simulink model "c00011M_harness"  (R2018a)
settings: Solver=FixedStepAuto  StartTime=0.0  StopTime=300  FixedStep=0.1  RelTol=1e-3
undefined symbols (not defined in the file): A1, hmax, PriorityTank, R1, R2, sigbuilder_block
(part 1 of 73)
settings Model: Creator=aarrieta  LastModifiedBy=umarkiegi

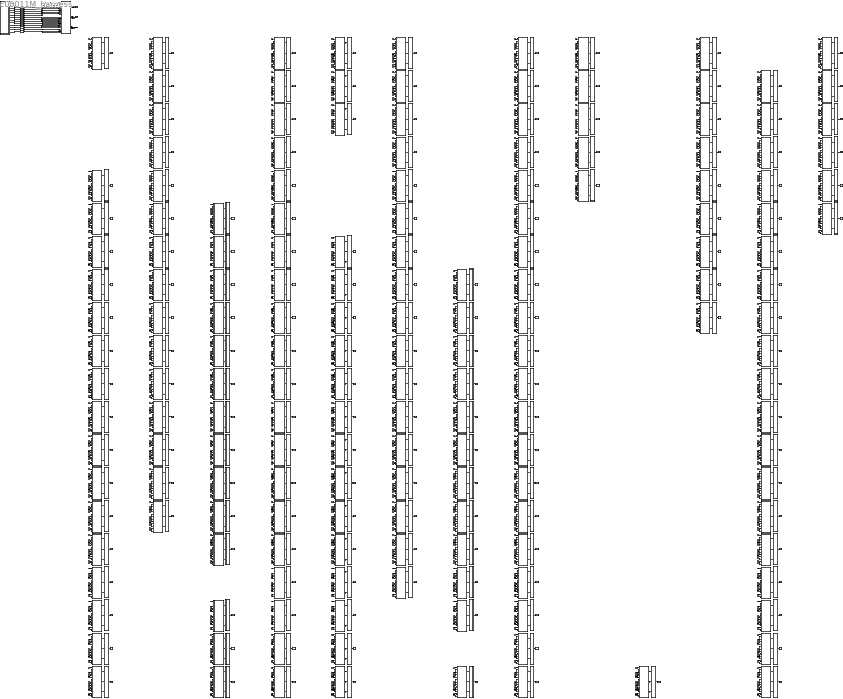
== system c00011M_harness ==
  CPSUT : Subsystem
  Eval : Subsystem
  Eval10 : Subsystem
  Eval100 : Subsystem
  Eval101 : Subsystem
  Eval102 : Subsystem
  Eval103 : Subsystem
  Eval104 : Subsystem
  Eval105 : Subsystem
  Eval106 : Subsystem
  Eval107 : Subsystem
  Eval108 : Subsystem
  Eval109 : Subsystem
  Eval11 : Subsystem
  Eval110 : Subsystem
  Eval111 : Subsystem
  Eval112 : Subsystem
  Eval113 : Subsystem
  Eval114 : Subsystem
  Eval115 : Subsystem
  Eval116 : Subsystem
  Eval12 : Subsystem
  Eval127 : Subsystem
  Eval128 : Subsystem
  Eval129 : Subsystem
  Eval13 : Subsystem
  Eval130 : Subsystem
  Eval131 : Subsystem
  Eval132 : Subsystem
  Eval133 : Subsystem
  Eval134 : Subsystem
  Eval135 : Subsystem
  Eval136 : Subsystem
  Eval137 : Subsystem
  Eval139 : Subsystem
  Eval14 : Subsystem
  Eval140 : Subsystem
  Eval141 : Subsystem
  Eval142 : Subsystem
  Eval143 : Subsystem
  Eval144 : Subsystem
  Eval145 : Subsystem
  Eval146 : Subsystem
  Eval147 : Subsystem
  Eval148 : Subsystem
  Eval149 : Subsystem
  Eval15 : Subsystem
  Eval150 : Subsystem
  Eval151 : Subsystem
  Eval152 : Subsystem
  Eval153 : Subsystem
  Eval154 : Subsystem
  Eval155 : Subsystem
  Eval156 : Subsystem
  Eval157 : Subsystem
  Eval158 : Subsystem
  Eval159 : Subsystem
  Eval16 : Subsystem
  Eval160 : Subsystem
  Eval161 : Subsystem
  Eval162 : Subsystem
  Eval163 : Subsystem
  Eval164 : Subsystem
  Eval17 : Subsystem
  Eval18 : Subsystem
  Eval19 : Subsystem
  Eval199 : Subsystem
  Eval20 : Subsystem
  Eval200 : Subsystem
  Eval201 : Subsystem
  Eval202 : Subsystem
  Eval203 : Subsystem
  Eval204 : Subsystem
  Eval205 : Subsystem
  Eval206 : Subsystem
  Eval207 : Subsystem
  Eval208 : Subsystem
  Eval21 : Subsystem
  Eval22 : Subsystem
  Eval221 : Subsystem
  Eval222 : Subsystem
  Eval223 : Subsystem
  Eval224 : Subsystem
  Eval225 : Subsystem
  Eval226 : Subsystem
  Eval227 : Subsystem
  Eval228 : Subsystem
  Eval229 : Subsystem
  Eval23 : Subsystem
  Eval230 : Subsystem
  Eval231 : Subsystem
  Eval232 : Subsystem
  Eval233 : Subsystem
  Eval234 : Subsystem
  Eval235 : Subsystem
  Eval236 : Subsystem
  Eval237 : Subsystem
  Eval238 : Subsystem
  Eval239 : Subsystem
  Eval24 : Subsystem
  Eval240 : Subsystem
  Eval241 : Subsystem
  Eval242 : Subsystem
  Eval243 : Subsystem
  Eval244 : Subsystem
  Eval245 : Subsystem
  Eval25 : Subsystem
  Eval26 : Subsystem
  Eval27 : Subsystem
  Eval28 : Subsystem
  Eval29 : Subsystem
  Eval30 : Subsystem
  Eval31 : Subsystem
  Eval32 : Subsystem
  Eval33 : Subsystem
  Eval34 : Subsystem
  Eval4 : Subsystem
  Eval45 : Subsystem
  Eval46 : Subsystem
  Eval47 : Subsystem
  Eval48 : Subsystem
  Eval49 : Subsystem
  Eval5 : Subsystem
  Eval50 : Subsystem
  Eval51 : Subsystem
  Eval52 : Subsystem
  Eval53 : Subsystem
  Eval54 : Subsystem
  Eval55 : Subsystem
  Eval57 : Subsystem
  Eval58 : Subsystem
  Eval59 : Subsystem
  Eval6 : Subsystem
  Eval60 : Subsystem
  Eval61 : Subsystem
  Eval62 : Subsystem
  Eval63 : Subsystem
  Eval64 : Subsystem
  Eval65 : Subsystem
  Eval66 : Subsystem
  Eval67 : Subsystem
  Eval68 : Subsystem
  Eval69 : Subsystem
  Eval7 : Subsystem
  Eval70 : Subsystem
  Eval71 : Subsystem
  Eval72 : Subsystem
  Eval73 : Subsystem
  Eval74 : Subsystem
  Eval75 : Subsystem
  Eval76 : Subsystem
  Eval77 : Subsystem
  Eval78 : Subsystem
  Eval79 : Subsystem
  Eval8 : Subsystem
  Eval80 : Subsystem
  Eval81 : Subsystem
  Eval82 : Subsystem
  Eval86 : Subsystem
  Eval87 : Subsystem
  Eval88 : Subsystem
  Eval89 : Subsystem
  Eval9 : Subsystem
  Eval90 : Subsystem
  Eval91 : Subsystem
  Eval92 : Subsystem
  Eval93 : Subsystem
  Eval94 : Subsystem
  Eval95 : Subsystem
  Eval96 : Subsystem
  Eval97 : Subsystem
  Eval98 : Subsystem
  Eval99 : Subsystem
  Inputs : Subsystem  Tag=STV Subsys  LoadFcn=sigbuilder_block('load');  StartFcn=sigbuilder_block('start');  StopFcn=sigbuilder_block('stop');  ClipboardFcn=sigbuilder_block('clipboard');  mask(Sigbuilder block){tuvar=[0:10]}
      mask init:
      | if ~strcmp(get_param(bdroot(gcb),'SimulationStatus'),'stopped'),tuvar = sigbuilder_block('maskInit'); end
      settings: CopyFcn=sigbuilder_block('copy');  DeleteFcn=sigbuilder_block('delete');  ModelCloseFcn=sigbuilder_block('modelClose');  PreSaveFcn=sigbuilder_block('preSave');  PauseFcn=sigbuilder_block('pause');  ContinueFcn=sigbuilder_block('continue');  NameChangeFcn=sigbuilder_block('namechange');  OpenFcn=sigbuilder_block('open',[276.75 163.5 675.75 486.75 ]);  CloseFcn=sigbuilder_block('close');
      mask Display: plot(0, 0, 100, 100,[2, 2, 32, 32, 2], [68, 8, 8, 68, 68],[32, 2], [38, 38], [32, 19, 2],[53, 60, 44], [32, 17, 17, 2],[16, 16, 31, 31]);txt = getActiveGroup(gcbh);text(2, 100, txt,'verticalAlignment', 'top');
  M001 : Subsystem
  M005 : Subsystem
  M006 : Subsystem
  M007 : Subsystem
  M008 : Subsystem
  M009 : Subsystem
  M010 : Subsystem
  M011 : Subsystem
  M012 : Subsystem
  M013 : Subsystem
  M014 : Subsystem
  M015 : Subsystem
  M016 : Subsystem
  M017 : Subsystem
  M018 : Subsystem
  M019 : Subsystem
  M020 : Subsystem
  M021 : Subsystem
  M022 : Subsystem
  M023 : Subsystem
  M024 : Subsystem
  M025 : Subsystem
  M026 : Subsystem
  M027 : Subsystem
  M028 : Subsystem
  M029 : Subsystem
  M030 : Subsystem
  M031 : Subsystem
  M032 : Subsystem
  M033 : Subsystem
  M034 : Subsystem
  M035 : Subsystem
  M046 : Subsystem
  M047 : Subsystem
  M048 : Subsystem
  M049 : Subsystem
  M050 : Subsystem
  M051 : Subsystem
  M052 : Subsystem
  M053 : Subsystem
  M054 : Subsystem
  M055 : Subsystem
  M056 : Subsystem
  M058 : Subsystem
  M059 : Subsystem
  M060 : Subsystem
  M061 : Subsystem
  M062 : Subsystem
  M063 : Subsystem
  M064 : Subsystem
  M065 : Subsystem
  M066 : Subsystem
  M067 : Subsystem
  M068 : Subsystem
  M069 : Subsystem
  M070 : Subsystem
  M071 : Subsystem
  M072 : Subsystem
  M073 : Subsystem
  M074 : Subsystem
  M075 : Subsystem
  M076 : Subsystem
  M077 : Subsystem
  M078 : Subsystem
  M079 : Subsystem
  M080 : Subsystem
  M081 : Subsystem
  M082 : Subsystem
  M083 : Subsystem
  M087 : Subsystem
  M088 : Subsystem
  M089 : Subsystem
  M090 : Subsystem
  M091 : Subsystem
  M092 : Subsystem
  M093 : Subsystem
  M094 : Subsystem
  M095 : Subsystem
  M096 : Subsystem
  M097 : Subsystem
  M098 : Subsystem
  M099 : Subsystem
  M100 : Subsystem
  M101 : Subsystem
  M102 : Subsystem
  M103 : Subsystem
  M104 : Subsystem
  M105 : Subsystem
  M106 : Subsystem
  M107 : Subsystem
  M108 : Subsystem
  M109 : Subsystem
  M110 : Subsystem
  M111 : Subsystem
  M112 : Subsystem
  M113 : Subsystem
  M114 : Subsystem
  M115 : Subsystem
  M116 : Subsystem
  M117 : Subsystem
  M128 : Subsystem
  M129 : Subsystem
  M130 : Subsystem
  M131 : Subsystem
  M132 : Subsystem
  M133 : Subsystem
  M134 : Subsystem
  M135 : Subsystem
  M136 : Subsystem
  M137 : Subsystem
  M138 : Subsystem
  M140 : Subsystem
  M141 : Subsystem
  M142 : Subsystem
  M143 : Subsystem
  M144 : Subsystem
  M145 : Subsystem
  M146 : Subsystem
  M147 : Subsystem
  M148 : Subsystem
  M149 : Subsystem
  M150 : Subsystem
  M151 : Subsystem
  M152 : Subsystem
  M153 : Subsystem
  M154 : Subsystem
  M155 : Subsystem
  M156 : Subsystem
  M157 : Subsystem
  M158 : Subsystem
  M159 : Subsystem
  M160 : Subsystem
  M161 : Subsystem
  M162 : Subsystem
  M163 : Subsystem
  M164 : Subsystem
  M165 : Subsystem
  M200 : Subsystem
  M201 : Subsystem
  M202 : Subsystem
  M203 : Subsystem
  M204 : Subsystem
  M205 : Subsystem
  M206 : Subsystem
  M207 : Subsystem
  M208 : Subsystem
  M209 : Subsystem
  M222 : Subsystem
  M223 : Subsystem
  M224 : Subsystem
  M225 : Subsystem
  M226 : Subsystem
  M227 : Subsystem
  M228 : Subsystem
  M229 : Subsystem
  M230 : Subsystem
  M231 : Subsystem
  M232 : Subsystem
  M233 : Subsystem
  M234 : Subsystem
  M235 : Subsystem
  M236 : Subsystem
  M237 : Subsystem
  M238 : Subsystem
  M239 : Subsystem
  M240 : Subsystem
  M241 : Subsystem
  M242 : Subsystem
  M243 : Subsystem
  M244 : Subsystem
  M245 : Subsystem
  M246 : Subsystem
  To Workspace : ToWorkspace  VariableName=mutant001  SampleTime=-1
  To Workspace10 : ToWorkspace  VariableName=mutant011  SampleTime=-1
  To Workspace100 : ToWorkspace  VariableName=mutant101  SampleTime=-1
  To Workspace101 : ToWorkspace  VariableName=mutant102  SampleTime=-1
  To Workspace102 : ToWorkspace  VariableName=mutant103  SampleTime=-1
  To Workspace103 : ToWorkspace  VariableName=mutant104  SampleTime=-1
  To Workspace104 : ToWorkspace  VariableName=mutant105  SampleTime=-1
  To Workspace105 : ToWorkspace  VariableName=mutant106  SampleTime=-1
  To Workspace106 : ToWorkspace  VariableName=mutant107  SampleTime=-1
  To Workspace107 : ToWorkspace  VariableName=mutant108  SampleTime=-1
  To Workspace108 : ToWorkspace  VariableName=mutant109  SampleTime=-1
  To Workspace109 : ToWorkspace  VariableName=mutant110  SampleTime=-1
  To Workspace11 : ToWorkspace  VariableName=mutant012  SampleTime=-1
  To Workspace110 : ToWorkspace  VariableName=mutant111  SampleTime=-1
  To Workspace111 : ToWorkspace  VariableName=mutant112  SampleTime=-1
  To Workspace112 : ToWorkspace  VariableName=mutant113  SampleTime=-1
  To Workspace113 : ToWorkspace  VariableName=mutant114  SampleTime=-1
  To Workspace114 : ToWorkspace  VariableName=mutant115  SampleTime=-1
  To Workspace115 : ToWorkspace  VariableName=mutant116  SampleTime=-1
  To Workspace116 : ToWorkspace  VariableName=mutant117  SampleTime=-1
  To Workspace12 : ToWorkspace  VariableName=mutant013  SampleTime=-1
  To Workspace127 : ToWorkspace  VariableName=mutant128  SampleTime=-1
  To Workspace128 : ToWorkspace  VariableName=mutant129  SampleTime=-1
  To Workspace129 : ToWorkspace  VariableName=mutant130  SampleTime=-1
  To Workspace13 : ToWorkspace  VariableName=mutant014  SampleTime=-1
  To Workspace130 : ToWorkspace  VariableName=mutant131  SampleTime=-1
  To Workspace131 : ToWorkspace  VariableName=mutant132  SampleTime=-1
  To Workspace132 : ToWorkspace  VariableName=mutant133  SampleTime=-1
  To Workspace133 : ToWorkspace  VariableName=mutant134  SampleTime=-1
  To Workspace134 : ToWorkspace  VariableName=mutant135  SampleTime=-1
  To Workspace135 : ToWorkspace  VariableName=mutant136  SampleTime=-1
  To Workspace136 : ToWorkspace  VariableName=mutant137  SampleTime=-1
  To Workspace137 : ToWorkspace  VariableName=mutant138  SampleTime=-1
  To Workspace139 : ToWorkspace  VariableName=mutant140  SampleTime=-1
  To Workspace14 : ToWorkspace  VariableName=mutant015  SampleTime=-1
  To Workspace140 : ToWorkspace  VariableName=mutant141  SampleTime=-1
  To Workspace141 : ToWorkspace  VariableName=mutant142  SampleTime=-1
  To Workspace142 : ToWorkspace  VariableName=mutant143  SampleTime=-1
  To Workspace143 : ToWorkspace  VariableName=mutant144  SampleTime=-1
  To Workspace144 : ToWorkspace  VariableName=mutant145  SampleTime=-1
  To Workspace145 : ToWorkspace  VariableName=mutant146  SampleTime=-1
  To Workspace146 : ToWorkspace  VariableName=mutant147  SampleTime=-1
  To Workspace147 : ToWorkspace  VariableName=mutant148  SampleTime=-1
  To Workspace148 : ToWorkspace  VariableName=mutant149  SampleTime=-1
  To Workspace149 : ToWorkspace  VariableName=mutant150  SampleTime=-1
  To Workspace15 : ToWorkspace  VariableName=mutant016  SampleTime=-1
  To Workspace150 : ToWorkspace  VariableName=mutant151  SampleTime=-1
  To Workspace151 : ToWorkspace  VariableName=mutant152  SampleTime=-1
  To Workspace152 : ToWorkspace  VariableName=mutant153  SampleTime=-1
  To Workspace153 : ToWorkspace  VariableName=mutant154  SampleTime=-1
  To Workspace154 : ToWorkspace  VariableName=mutant155  SampleTime=-1
  To Workspace155 : ToWorkspace  VariableName=mutant156  SampleTime=-1
  To Workspace156 : ToWorkspace  VariableName=mutant157  SampleTime=-1
  To Workspace157 : ToWorkspace  VariableName=mutant158  SampleTime=-1
  To Workspace158 : ToWorkspace  VariableName=mutant159  SampleTime=-1
  To Workspace159 : ToWorkspace  VariableName=mutant160  SampleTime=-1
  To Workspace16 : ToWorkspace  VariableName=mutant017  SampleTime=-1
  To Workspace160 : ToWorkspace  VariableName=mutant161  SampleTime=-1
  To Workspace161 : ToWorkspace  VariableName=mutant162  SampleTime=-1
  To Workspace162 : ToWorkspace  VariableName=mutant163  SampleTime=-1
  To Workspace163 : ToWorkspace  VariableName=mutant164  SampleTime=-1
  To Workspace164 : ToWorkspace  VariableName=mutant165  SampleTime=-1
  To Workspace17 : ToWorkspace  VariableName=mutant018  SampleTime=-1
  To Workspace18 : ToWorkspace  VariableName=mutant019  SampleTime=-1
  To Workspace19 : ToWorkspace  VariableName=mutant020  SampleTime=-1
  To Workspace199 : ToWorkspace  VariableName=mutant200  SampleTime=-1
  To Workspace20 : ToWorkspace  VariableName=mutant021  SampleTime=-1
  To Workspace200 : ToWorkspace  VariableName=mutant201  SampleTime=-1
  To Workspace201 : ToWorkspace  VariableName=mutant202  SampleTime=-1
  To Workspace202 : ToWorkspace  VariableName=mutant203  SampleTime=-1
  To Workspace203 : ToWorkspace  VariableName=mutant204  SampleTime=-1
  To Workspace204 : ToWorkspace  VariableName=mutant205  SampleTime=-1
  To Workspace205 : ToWorkspace  VariableName=mutant206  SampleTime=-1
  To Workspace206 : ToWorkspace  VariableName=mutant207  SampleTime=-1
  To Workspace207 : ToWorkspace  VariableName=mutant208  SampleTime=-1
  To Workspace208 : ToWorkspace  VariableName=mutant209  SampleTime=-1
  To Workspace21 : ToWorkspace  VariableName=mutant022  SampleTime=-1
  To Workspace22 : ToWorkspace  VariableName=mutant023  SampleTime=-1
  To Workspace221 : ToWorkspace  VariableName=mutant222  SampleTime=-1
  To Workspace222 : ToWorkspace  VariableName=mutant223  SampleTime=-1
  To Workspace223 : ToWorkspace  VariableName=mutant224  SampleTime=-1
  To Workspace224 : ToWorkspace  VariableName=mutant225  SampleTime=-1
  To Workspace225 : ToWorkspace  VariableName=mutant226  SampleTime=-1
  To Workspace226 : ToWorkspace  VariableName=mutant227  SampleTime=-1
  To Workspace227 : ToWorkspace  VariableName=mutant228  SampleTime=-1
  To Workspace228 : ToWorkspace  VariableName=mutant229  SampleTime=-1
  To Workspace229 : ToWorkspace  VariableName=mutant230  SampleTime=-1
  To Workspace23 : ToWorkspace  VariableName=mutant024  SampleTime=-1
  To Workspace230 : ToWorkspace  VariableName=mutant231  SampleTime=-1
  To Workspace231 : ToWorkspace  VariableName=mutant232  SampleTime=-1
  To Workspace232 : ToWorkspace  VariableName=mutant233  SampleTime=-1
  To Workspace233 : ToWorkspace  VariableName=mutant234  SampleTime=-1
  To Workspace234 : ToWorkspace  VariableName=mutant235  SampleTime=-1
  To Workspace235 : ToWorkspace  VariableName=mutant236  SampleTime=-1
  To Workspace236 : ToWorkspace  VariableName=mutant237  SampleTime=-1
  To Workspace237 : ToWorkspace  VariableName=mutant238  SampleTime=-1
  To Workspace238 : ToWorkspace  VariableName=mutant239  SampleTime=-1
  To Workspace239 : ToWorkspace  VariableName=mutant240  SampleTime=-1
  To Workspace24 : ToWorkspace  VariableName=mutant025  SampleTime=-1
  To Workspace240 : ToWorkspace  VariableName=mutant241  SampleTime=-1
  To Workspace241 : ToWorkspace  VariableName=mutant242  SampleTime=-1
  To Workspace242 : ToWorkspace  VariableName=mutant243  SampleTime=-1
  To Workspace243 : ToWorkspace  VariableName=mutant244  SampleTime=-1
  To Workspace244 : ToWorkspace  VariableName=mutant245  SampleTime=-1
  To Workspace245 : ToWorkspace  VariableName=mutant246  SampleTime=-1
  To Workspace25 : ToWorkspace  VariableName=mutant026  SampleTime=-1
  To Workspace26 : ToWorkspace  VariableName=mutant027  SampleTime=-1
  To Workspace27 : ToWorkspace  VariableName=mutant028  SampleTime=-1
  To Workspace28 : ToWorkspace  VariableName=mutant029  SampleTime=-1
  To Workspace29 : ToWorkspace  VariableName=mutant030  SampleTime=-1
  To Workspace30 : ToWorkspace  VariableName=mutant031  SampleTime=-1
  To Workspace31 : ToWorkspace  VariableName=mutant032  SampleTime=-1
  To Workspace32 : ToWorkspace  VariableName=mutant033  SampleTime=-1
  To Workspace33 : ToWorkspace  VariableName=mutant034  SampleTime=-1
  To Workspace34 : ToWorkspace  VariableName=mutant035  SampleTime=-1
  To Workspace4 : ToWorkspace  VariableName=mutant005  SampleTime=-1
  To Workspace45 : ToWorkspace  VariableName=mutant046  SampleTime=-1
  To Workspace46 : ToWorkspace  VariableName=mutant047  SampleTime=-1
  To Workspace47 : ToWorkspace  VariableName=mutant048  SampleTime=-1
  To Workspace48 : ToWorkspace  VariableName=mutant049  SampleTime=-1
  To Workspace49 : ToWorkspace  VariableName=mutant050  SampleTime=-1
  To Workspace5 : ToWorkspace  VariableName=mutant006  SampleTime=-1
  To Workspace50 : ToWorkspace  VariableName=mutant051  SampleTime=-1
  To Workspace51 : ToWorkspace  VariableName=mutant052  SampleTime=-1
  To Workspace52 : ToWorkspace  VariableName=mutant053  SampleTime=-1
  To Workspace53 : ToWorkspace  VariableName=mutant054  SampleTime=-1
  To Workspace54 : ToWorkspace  VariableName=mutant055  SampleTime=-1
  To Workspace55 : ToWorkspace  VariableName=mutant056  SampleTime=-1
  To Workspace57 : ToWorkspace  VariableName=mutant058  SampleTime=-1
  To Workspace58 : ToWorkspace  VariableName=mutant059  SampleTime=-1
  To Workspace59 : ToWorkspace  VariableName=mutant060  SampleTime=-1
  To Workspace6 : ToWorkspace  VariableName=mutant007  SampleTime=-1
  To Workspace60 : ToWorkspace  VariableName=mutant061  SampleTime=-1
  To Workspace61 : ToWorkspace  VariableName=mutant062  SampleTime=-1
  To Workspace62 : ToWorkspace  VariableName=mutant063  SampleTime=-1
  To Workspace63 : ToWorkspace  VariableName=mutant064  SampleTime=-1
  To Workspace64 : ToWorkspace  VariableName=mutant065  SampleTime=-1
  To Workspace65 : ToWorkspace  VariableName=mutant066  SampleTime=-1
  To Workspace66 : ToWorkspace  VariableName=mutant067  SampleTime=-1
  To Workspace67 : ToWorkspace  VariableName=mutant068  SampleTime=-1
  To Workspace68 : ToWorkspace  VariableName=mutant069  SampleTime=-1
  To Workspace69 : ToWorkspace  VariableName=mutant070  SampleTime=-1
  To Workspace7 : ToWorkspace  VariableName=mutant008  SampleTime=-1
  To Workspace70 : ToWorkspace  VariableName=mutant071  SampleTime=-1
  To Workspace71 : ToWorkspace  VariableName=mutant072  SampleTime=-1
  To Workspace72 : ToWorkspace  VariableName=mutant073  SampleTime=-1
  To Workspace73 : ToWorkspace  VariableName=mutant074  SampleTime=-1
  To Workspace74 : ToWorkspace  VariableName=mutant075  SampleTime=-1
  To Workspace75 : ToWorkspace  VariableName=mutant076  SampleTime=-1
  To Workspace76 : ToWorkspace  VariableName=mutant077  SampleTime=-1
  To Workspace77 : ToWorkspace  VariableName=mutant078  SampleTime=-1
  To Workspace78 : ToWorkspace  VariableName=mutant079  SampleTime=-1
  To Workspace79 : ToWorkspace  VariableName=mutant080  SampleTime=-1
  To Workspace8 : ToWorkspace  VariableName=mutant009  SampleTime=-1
  To Workspace80 : ToWorkspace  VariableName=mutant081  SampleTime=-1
  To Workspace81 : ToWorkspace  VariableName=mutant082  SampleTime=-1
  To Workspace82 : ToWorkspace  VariableName=mutant083  SampleTime=-1
  To Workspace86 : ToWorkspace  VariableName=mutant087  SampleTime=-1
  To Workspace87 : ToWorkspace  VariableName=mutant088  SampleTime=-1
  To Workspace88 : ToWorkspace  VariableName=mutant089  SampleTime=-1
  To Workspace89 : ToWorkspace  VariableName=mutant090  SampleTime=-1
  To Workspace9 : ToWorkspace  VariableName=mutant010  SampleTime=-1
  To Workspace90 : ToWorkspace  VariableName=mutant091  SampleTime=-1
  To Workspace91 : ToWorkspace  VariableName=mutant092  SampleTime=-1
  To Workspace92 : ToWorkspace  VariableName=mutant093  SampleTime=-1
  To Workspace93 : ToWorkspace  VariableName=mutant094  SampleTime=-1
  To Workspace94 : ToWorkspace  VariableName=mutant095  SampleTime=-1
  To Workspace95 : ToWorkspace  VariableName=mutant096  SampleTime=-1
  To Workspace96 : ToWorkspace  VariableName=mutant097  SampleTime=-1
  To Workspace97 : ToWorkspace  VariableName=mutant098  SampleTime=-1
  To Workspace98 : ToWorkspace  VariableName=mutant099  SampleTime=-1
  To Workspace99 : ToWorkspace  VariableName=mutant100  SampleTime=-1
  dtc_CT1 : DataTypeConversion
  dtc_CT2 : DataTypeConversion
  dtc_CT3 : DataTypeConversion
  dtc_E3 : DataTypeConversion
  dtc_EB1 : DataTypeConversion
  dtc_EB2 : DataTypeConversion
  dtc_EB3 : DataTypeConversion
  dtc_F3 : DataTypeConversion
  dtc_MR1 : DataTypeConversion
  dtc_MR2 : DataTypeConversion
  dtc_T1 : DataTypeConversion
  dtc_T2 : DataTypeConversion
  dtc_T3 : DataTypeConversion
  LL1 : Outport
  LL2 : Outport  Port=2
  LL3 : Outport  Port=3
  tag scope: out1=global, out2=global, out3=global
  wires:
  CPSUT/1(LL1) -> [out1], LL1/1
  CPSUT/2(LL2) -> [out2], LL2/1
  CPSUT/3(LL3) -> [out3], LL3/1
  [in1] -> M001/1(CT1)
  [in4] -> M001/2(MR1)
  [in5] -> M001/3(T1)
  [in6] -> M001/4(EB1)
  [in7] -> M001/5(CT2)
  [in10] -> M001/6(MR2)
  [in11] -> M001/7(T2)
  [in12] -> M001/8(EB2)
  [in13] -> M001/9(CT3)
  [in14] -> M001/10(F3)
  [in15] -> M001/11(E3)
  [in17] -> M001/12(T3)
  [in18] -> M001/13(EB3)
  Eval/1(Out1) -> To Workspace/1
  M001/1(LL1) -> Eval/1(In1)
  M001/2(LL2) -> Eval/2(In2)
  M001/3(LL3) -> Eval/3(In3)
  [in1] -> M005/1(CT1)
  [in4] -> M005/2(MR1)
  [in5] -> M005/3(T1)
  [in6] -> M005/4(EB1)
  [in7] -> M005/5(CT2)
  [in10] -> M005/6(MR2)
  [in11] -> M005/7(T2)
  [in12] -> M005/8(EB2)
  [in13] -> M005/9(CT3)
  [in14] -> M005/10(F3)
  [in15] -> M005/11(E3)
  [in17] -> M005/12(T3)
  [in18] -> M005/13(EB3)
  M005/1(LL1) -> Eval4/1(In1)
  M005/2(LL2) -> Eval4/2(In2)
  M005/3(LL3) -> Eval4/3(In3)
  Eval4/1(Out1) -> To Workspace4/1
  [in1] -> M006/1(CT1)
  [in4] -> M006/2(MR1)
  [in5] -> M006/3(T1)
  [in6] -> M006/4(EB1)
  [in7] -> M006/5(CT2)
  [in10] -> M006/6(MR2)
  [in11] -> M006/7(T2)
  [in12] -> M006/8(EB2)
  [in13] -> M006/9(CT3)
  [in14] -> M006/10(F3)
  [in15] -> M006/11(E3)
  [in17] -> M006/12(T3)
  [in18] -> M006/13(EB3)
  M006/1(LL1) -> Eval5/1(In1)
  M006/2(LL2) -> Eval5/2(In2)
  M006/3(LL3) -> Eval5/3(In3)
  Eval5/1(Out1) -> To Workspace5/1
  [in1] -> M007/1(CT1)
  [in4] -> M007/2(MR1)
  [in5] -> M007/3(T1)
  [in6] -> M007/4(EB1)
  [in7] -> M007/5(CT2)
  [in10] -> M007/6(MR2)
  [in11] -> M007/7(T2)
  [in12] -> M007/8(EB2)
  [in13] -> M007/9(CT3)
  [in14] -> M007/10(F3)
  [in15] -> M007/11(E3)
  [in17] -> M007/12(T3)
  [in18] -> M007/13(EB3)
  M007/1(LL1) -> Eval6/1(In1)
  M007/2(LL2) -> Eval6/2(In2)
  M007/3(LL3) -> Eval6/3(In3)
  Eval6/1(Out1) -> To Workspace6/1
  [in1] -> M008/1(CT1)
  [in4] -> M008/2(MR1)
  [in5] -> M008/3(T1)
  [in6] -> M008/4(EB1)
  [in7] -> M008/5(CT2)
  [in10] -> M008/6(MR2)
  [in11] -> M008/7(T2)
  [in12] -> M008/8(EB2)
  [in13] -> M008/9(CT3)
  [in14] -> M008/10(F3)
  [in15] -> M008/11(E3)
  [in17] -> M008/12(T3)
  [in18] -> M008/13(EB3)
  M008/1(LL1) -> Eval7/1(In1)
  M008/2(LL2) -> Eval7/2(In2)
  M008/3(LL3) -> Eval7/3(In3)
  Eval7/1(Out1) -> To Workspace7/1
  [in1] -> M009/1(CT1)
  [in4] -> M009/2(MR1)
  [in5] -> M009/3(T1)
  [in6] -> M009/4(EB1)
  [in7] -> M009/5(CT2)
  [in10] -> M009/6(MR2)
  [in11] -> M009/7(T2)
  [in12] -> M009/8(EB2)
  [in13] -> M009/9(CT3)
  [in14] -> M009/10(F3)
  [in15] -> M009/11(E3)
  [in17] -> M009/12(T3)
  [in18] -> M009/13(EB3)
  M009/1(LL1) -> Eval8/1(In1)
  M009/2(LL2) -> Eval8/2(In2)
  M009/3(LL3) -> Eval8/3(In3)
  Eval8/1(Out1) -> To Workspace8/1
  [in1] -> M010/1(CT1)
  [in4] -> M010/2(MR1)
  [in5] -> M010/3(T1)
  [in6] -> M010/4(EB1)
  [in7] -> M010/5(CT2)
  [in10] -> M010/6(MR2)
  [in11] -> M010/7(T2)
  [in12] -> M010/8(EB2)
  [in13] -> M010/9(CT3)
  [in14] -> M010/10(F3)
  [in15] -> M010/11(E3)
  [in17] -> M010/12(T3)
  [in18] -> M010/13(EB3)
  M010/1(LL1) -> Eval9/1(In1)
  M010/2(LL2) -> Eval9/2(In2)
  M010/3(LL3) -> Eval9/3(In3)
  Eval9/1(Out1) -> To Workspace9/1
  [in1] -> M011/1(CT1)
  [in4] -> M011/2(MR1)
  [in5] -> M011/3(T1)
  [in6] -> M011/4(EB1)
  [in7] -> M011/5(CT2)
  [in10] -> M011/6(MR2)
  [in11] -> M011/7(T2)
  [in12] -> M011/8(EB2)
  [in13] -> M011/9(CT3)
  [in14] -> M011/10(F3)
  [in15] -> M011/11(E3)
  [in17] -> M011/12(T3)
  [in18] -> M011/13(EB3)
  M011/1(LL1) -> Eval10/1(In1)
  M011/2(LL2) -> Eval10/2(In2)
  M011/3(LL3) -> Eval10/3(In3)
  Eval10/1(Out1) -> To Workspace10/1
  [in1] -> M012/1(CT1)
  [in4] -> M012/2(MR1)
  [in5] -> M012/3(T1)
  [in6] -> M012/4(EB1)
  [in7] -> M012/5(CT2)
  [in10] -> M012/6(MR2)
  [in11] -> M012/7(T2)
  [in12] -> M012/8(EB2)
  [in13] -> M012/9(CT3)
  [in14] -> M012/10(F3)
  [in15] -> M012/11(E3)
  [in17] -> M012/12(T3)
  [in18] -> M012/13(EB3)
  M012/1(LL1) -> Eval11/1(In1)
  M012/2(LL2) -> Eval11/2(In2)
  M012/3(LL3) -> Eval11/3(In3)
  Eval11/1(Out1) -> To Workspace11/1
  [in1] -> M013/1(CT1)
  [in4] -> M013/2(MR1)
  [in5] -> M013/3(T1)
  [in6] -> M013/4(EB1)
  [in7] -> M013/5(CT2)
  [in10] -> M013/6(MR2)
  [in11] -> M013/7(T2)
  [in12] -> M013/8(EB2)
  [in13] -> M013/9(CT3)
  [in14] -> M013/10(F3)
  [in15] -> M013/11(E3)
  [in17] -> M013/12(T3)
  [in18] -> M013/13(EB3)
  M013/1(LL1) -> Eval12/1(In1)
  M013/2(LL2) -> Eval12/2(In2)
  M013/3(LL3) -> Eval12/3(In3)
  Eval12/1(Out1) -> To Workspace12/1
  [in1] -> M014/1(CT1)
  [in4] -> M014/2(MR1)
  [in5] -> M014/3(T1)
  [in6] -> M014/4(EB1)
  [in7] -> M014/5(CT2)
  [in10] -> M014/6(MR2)
  [in11] -> M014/7(T2)
  [in12] -> M014/8(EB2)
  [in13] -> M014/9(CT3)
  [in14] -> M014/10(F3)
  [in15] -> M014/11(E3)
  [in17] -> M014/12(T3)
  [in18] -> M014/13(EB3)
  M014/1(LL1) -> Eval13/1(In1)
  M014/2(LL2) -> Eval13/2(In2)
  M014/3(LL3) -> Eval13/3(In3)
  Eval13/1(Out1) -> To Workspace13/1
  [in1] -> M015/1(CT1)
  [in4] -> M015/2(MR1)
  [in5] -> M015/3(T1)
  [in6] -> M015/4(EB1)
  [in7] -> M015/5(CT2)
  [in10] -> M015/6(MR2)
  [in11] -> M015/7(T2)
  [in12] -> M015/8(EB2)
  [in13] -> M015/9(CT3)
  [in14] -> M015/10(F3)
  [in15] -> M015/11(E3)
  [in17] -> M015/12(T3)
  [in18] -> M015/13(EB3)
  M015/1(LL1) -> Eval14/1(In1)
  M015/2(LL2) -> Eval14/2(In2)
  M015/3(LL3) -> Eval14/3(In3)
  Eval14/1(Out1) -> To Workspace14/1
  [in1] -> M016/1(CT1)
  [in4] -> M016/2(MR1)
  [in5] -> M016/3(T1)
  [in6] -> M016/4(EB1)
  [in7] -> M016/5(CT2)
  [in10] -> M016/6(MR2)
  [in11] -> M016/7(T2)
  [in12] -> M016/8(EB2)
  [in13] -> M016/9(CT3)
  [in14] -> M016/10(F3)
  [in15] -> M016/11(E3)
  [in17] -> M016/12(T3)
  [in18] -> M016/13(EB3)
  M016/1(LL1) -> Eval15/1(In1)
  M016/2(LL2) -> Eval15/2(In2)
  M016/3(LL3) -> Eval15/3(In3)
  Eval15/1(Out1) -> To Workspace15/1
  [in1] -> M017/1(CT1)
  [in4] -> M017/2(MR1)
  [in5] -> M017/3(T1)
  [in6] -> M017/4(EB1)
  [in7] -> M017/5(CT2)
  [in10] -> M017/6(MR2)
  [in11] -> M017/7(T2)
  [in12] -> M017/8(EB2)
  [in13] -> M017/9(CT3)
  [in14] -> M017/10(F3)
  [in15] -> M017/11(E3)
  [in17] -> M017/12(T3)
  [in18] -> M017/13(EB3)
  M017/1(LL1) -> Eval16/1(In1)
  M017/2(LL2) -> Eval16/2(In2)
  M017/3(LL3) -> Eval16/3(In3)
  Eval16/1(Out1) -> To Workspace16/1
  [in1] -> M018/1(CT1)
  [in4] -> M018/2(MR1)
  [in5] -> M018/3(T1)
  [in6] -> M018/4(EB1)
  [in7] -> M018/5(CT2)
  [in10] -> M018/6(MR2)
  [in11] -> M018/7(T2)
  [in12] -> M018/8(EB2)
  [in13] -> M018/9(CT3)
  [in14] -> M018/10(F3)
  [in15] -> M018/11(E3)
  [in17] -> M018/12(T3)
  [in18] -> M018/13(EB3)
  M018/1(LL1) -> Eval17/1(In1)
  M018/2(LL2) -> Eval17/2(In2)
  M018/3(LL3) -> Eval17/3(In3)
  Eval17/1(Out1) -> To Workspace17/1
  [in1] -> M019/1(CT1)
  [in4] -> M019/2(MR1)
  [in5] -> M019/3(T1)
  [in6] -> M019/4(EB1)
  [in7] -> M019/5(CT2)
  [in10] -> M019/6(MR2)
  [in11] -> M019/7(T2)
  [in12] -> M019/8(EB2)
  [in13] -> M019/9(CT3)
  [in14] -> M019/10(F3)
  [in15] -> M019/11(E3)
  [in17] -> M019/12(T3)
  [in18] -> M019/13(EB3)
  M019/1(LL1) -> Eval18/1(In1)
  M019/2(LL2) -> Eval18/2(In2)
  M019/3(LL3) -> Eval18/3(In3)
  Eval18/1(Out1) -> To Workspace18/1
  [in1] -> M020/1(CT1)
  [in4] -> M020/2(MR1)
  [in5] -> M020/3(T1)
  [in6] -> M020/4(EB1)
  [in7] -> M020/5(CT2)
  [in10] -> M020/6(MR2)
  [in11] -> M020/7(T2)
  [in12] -> M020/8(EB2)
  [in13] -> M020/9(CT3)
  [in14] -> M020/10(F3)
  [in15] -> M020/11(E3)
  [in17] -> M020/12(T3)
  [in18] -> M020/13(EB3)
  M020/1(LL1) -> Eval19/1(In1)
  M020/2(LL2) -> Eval19/2(In2)
  M020/3(LL3) -> Eval19/3(In3)
  Eval19/1(Out1) -> To Workspace19/1
  [in1] -> M021/1(CT1)
  [in4] -> M021/2(MR1)
  [in5] -> M021/3(T1)
  [in6] -> M021/4(EB1)
  [in7] -> M021/5(CT2)
  [in10] -> M021/6(MR2)
  [in11] -> M021/7(T2)
  [in12] -> M021/8(EB2)
  [in13] -> M021/9(CT3)
  [in14] -> M021/10(F3)
  [in15] -> M021/11(E3)
  [in17] -> M021/12(T3)
  [in18] -> M021/13(EB3)
  M021/1(LL1) -> Eval20/1(In1)
  M021/2(LL2) -> Eval20/2(In2)
  M021/3(LL3) -> Eval20/3(In3)
  Eval20/1(Out1) -> To Workspace20/1
  [in1] -> M022/1(CT1)
  [in4] -> M022/2(MR1)
  [in5] -> M022/3(T1)
  [in6] -> M022/4(EB1)
  [in7] -> M022/5(CT2)
  [in10] -> M022/6(MR2)
  [in11] -> M022/7(T2)
  [in12] -> M022/8(EB2)
  [in13] -> M022/9(CT3)
  [in14] -> M022/10(F3)
  [in15] -> M022/11(E3)
  [in17] -> M022/12(T3)
  [in18] -> M022/13(EB3)
  M022/1(LL1) -> Eval21/1(In1)
  M022/2(LL2) -> Eval21/2(In2)
  M022/3(LL3) -> Eval21/3(In3)
  Eval21/1(Out1) -> To Workspace21/1
  [in1] -> M023/1(CT1)
  [in4] -> M023/2(MR1)
  [in5] -> M023/3(T1)
  [in6] -> M023/4(EB1)
  [in7] -> M023/5(CT2)
  [in10] -> M023/6(MR2)
  [in11] -> M023/7(T2)
  [in12] -> M023/8(EB2)
  [in13] -> M023/9(CT3)
  [in14] -> M023/10(F3)
  [in15] -> M023/11(E3)
  [in17] -> M023/12(T3)
  [in18] -> M023/13(EB3)
  M023/1(LL1) -> Eval22/1(In1)
  M023/2(LL2) -> Eval22/2(In2)
  M023/3(LL3) -> Eval22/3(In3)
  Eval22/1(Out1) -> To Workspace22/1
  [in1] -> M024/1(CT1)
  [in4] -> M024/2(MR1)
  [in5] -> M024/3(T1)
  [in6] -> M024/4(EB1)
  [in7] -> M024/5(CT2)
  [in10] -> M024/6(MR2)
  [in11] -> M024/7(T2)
  [in12] -> M024/8(EB2)
  [in13] -> M024/9(CT3)
  [in14] -> M024/10(F3)
  [in15] -> M024/11(E3)
  [in17] -> M024/12(T3)
  [in18] -> M024/13(EB3)
  M024/1(LL1) -> Eval23/1(In1)
  M024/2(LL2) -> Eval23/2(In2)
  M024/3(LL3) -> Eval23/3(In3)
  Eval23/1(Out1) -> To Workspace23/1
  [in1] -> M025/1(CT1)
  [in4] -> M025/2(MR1)
  [in5] -> M025/3(T1)
  [in6] -> M025/4(EB1)
  [in7] -> M025/5(CT2)
  [in10] -> M025/6(MR2)
  [in11] -> M025/7(T2)
  [in12] -> M025/8(EB2)
  [in13] -> M025/9(CT3)
  [in14] -> M025/10(F3)
  [in15] -> M025/11(E3)
  [in17] -> M025/12(T3)
  [in18] -> M025/13(EB3)
  M025/1(LL1) -> Eval24/1(In1)
  M025/2(LL2) -> Eval24/2(In2)
  M025/3(LL3) -> Eval24/3(In3)
  Eval24/1(Out1) -> To Workspace24/1
  [in1] -> M026/1(CT1)
  [in4] -> M026/2(MR1)
  [in5] -> M026/3(T1)
  [in6] -> M026/4(EB1)
  [in7] -> M026/5(CT2)
  [in10] -> M026/6(MR2)
  [in11] -> M026/7(T2)
  [in12] -> M026/8(EB2)
  [in13] -> M026/9(CT3)
  [in14] -> M026/10(F3)
  [in15] -> M026/11(E3)
  [in17] -> M026/12(T3)
  [in18] -> M026/13(EB3)
  M026/1(LL1) -> Eval25/1(In1)
  M026/2(LL2) -> Eval25/2(In2)
  M026/3(LL3) -> Eval25/3(In3)
  Eval25/1(Out1) -> To Workspace25/1
  [in1] -> M027/1(CT1)
  [in4] -> M027/2(MR1)
  [in5] -> M027/3(T1)
  [in6] -> M027/4(EB1)
  [in7] -> M027/5(CT2)
  [in10] -> M027/6(MR2)
  [in11] -> M027/7(T2)
  [in12] -> M027/8(EB2)
  [in13] -> M027/9(CT3)
  [in14] -> M027/10(F3)
  [in15] -> M027/11(E3)
  [in17] -> M027/12(T3)
  [in18] -> M027/13(EB3)
  M027/1(LL1) -> Eval26/1(In1)
  M027/2(LL2) -> Eval26/2(In2)
  M027/3(LL3) -> Eval26/3(In3)
  Eval26/1(Out1) -> To Workspace26/1
  [in1] -> M028/1(CT1)
  [in4] -> M028/2(MR1)
  [in5] -> M028/3(T1)
  [in6] -> M028/4(EB1)
  [in7] -> M028/5(CT2)
  [in10] -> M028/6(MR2)
  [in11] -> M028/7(T2)
  [in12] -> M028/8(EB2)
  [in13] -> M028/9(CT3)
  [in14] -> M028/10(F3)
  [in15] -> M028/11(E3)
  [in17] -> M028/12(T3)
  [in18] -> M028/13(EB3)
  M028/1(LL1) -> Eval27/1(In1)
  M028/2(LL2) -> Eval27/2(In2)
  M028/3(LL3) -> Eval27/3(In3)
  Eval27/1(Out1) -> To Workspace27/1
  [in1] -> M029/1(CT1)
  [in4] -> M029/2(MR1)
  [in5] -> M029/3(T1)
  [in6] -> M029/4(EB1)
  [in7] -> M029/5(CT2)
  [in10] -> M029/6(MR2)
  [in11] -> M029/7(T2)
  [in12] -> M029/8(EB2)
  [in13] -> M029/9(CT3)
  [in14] -> M029/10(F3)
  [in15] -> M029/11(E3)
  [in17] -> M029/12(T3)
  [in18] -> M029/13(EB3)
  M029/1(LL1) -> Eval28/1(In1)
  M029/2(LL2) -> Eval28/2(In2)
  M029/3(LL3) -> Eval28/3(In3)
  Eval28/1(Out1) -> To Workspace28/1
  [in1] -> M030/1(CT1)
  [in4] -> M030/2(MR1)
  [in5] -> M030/3(T1)
  [in6] -> M030/4(EB1)
  [in7] -> M030/5(CT2)
  [in10] -> M030/6(MR2)
  [in11] -> M030/7(T2)
  [in12] -> M030/8(EB2)
  [in13] -> M030/9(CT3)
  [in14] -> M030/10(F3)
  [in15] -> M030/11(E3)
  [in17] -> M030/12(T3)
  [in18] -> M030/13(EB3)
  M030/1(LL1) -> Eval29/1(In1)
  M030/2(LL2) -> Eval29/2(In2)
  M030/3(LL3) -> Eval29/3(In3)
  Eval29/1(Out1) -> To Workspace29/1
  [in1] -> M031/1(CT1)
  [in4] -> M031/2(MR1)
  [in5] -> M031/3(T1)
  [in6] -> M031/4(EB1)
  [in7] -> M031/5(CT2)
  [in10] -> M031/6(MR2)
  [in11] -> M031/7(T2)
  [in12] -> M031/8(EB2)
  [in13] -> M031/9(CT3)
  [in14] -> M031/10(F3)
  [in15] -> M031/11(E3)
  [in17] -> M031/12(T3)
  [in18] -> M031/13(EB3)
  M031/1(LL1) -> Eval30/1(In1)
  M031/2(LL2) -> Eval30/2(In2)
  M031/3(LL3) -> Eval30/3(In3)
  Eval30/1(Out1) -> To Workspace30/1
  [in1] -> M032/1(CT1)
  [in4] -> M032/2(MR1)
  [in5] -> M032/3(T1)
  [in6] -> M032/4(EB1)
  [in7] -> M032/5(CT2)
  [in10] -> M032/6(MR2)
  [in11] -> M032/7(T2)
  [in12] -> M032/8(EB2)
  [in13] -> M032/9(CT3)
  [in14] -> M032/10(F3)
  [in15] -> M032/11(E3)
  [in17] -> M032/12(T3)
  [in18] -> M032/13(EB3)
  M032/1(LL1) -> Eval31/1(In1)
  M032/2(LL2) -> Eval31/2(In2)
  M032/3(LL3) -> Eval31/3(In3)
  Eval31/1(Out1) -> To Workspace31/1
  [in1] -> M033/1(CT1)
  [in4] -> M033/2(MR1)
  [in5] -> M033/3(T1)
  [in6] -> M033/4(EB1)
  [in7] -> M033/5(CT2)
  [in10] -> M033/6(MR2)
  [in11] -> M033/7(T2)
  [in12] -> M033/8(EB2)
  [in13] -> M033/9(CT3)
  [in14] -> M033/10(F3)
  [in15] -> M033/11(E3)
  [in17] -> M033/12(T3)
  [in18] -> M033/13(EB3)
  M033/1(LL1) -> Eval32/1(In1)
  M033/2(LL2) -> Eval32/2(In2)
  M033/3(LL3) -> Eval32/3(In3)
  Eval32/1(Out1) -> To Workspace32/1
  [in1] -> M034/1(CT1)
  [in4] -> M034/2(MR1)
  [in5] -> M034/3(T1)
  [in6] -> M034/4(EB1)
  [in7] -> M034/5(CT2)
  [in10] -> M034/6(MR2)
  [in11] -> M034/7(T2)
  [in12] -> M034/8(EB2)
  [in13] -> M034/9(CT3)
  [in14] -> M034/10(F3)
  [in15] -> M034/11(E3)
  [in17] -> M034/12(T3)
  [in18] -> M034/13(EB3)
  M034/1(LL1) -> Eval33/1(In1)
  M034/2(LL2) -> Eval33/2(In2)
  M034/3(LL3) -> Eval33/3(In3)
  Eval33/1(Out1) -> To Workspace33/1
  [in1] -> M035/1(CT1)
  [in4] -> M035/2(MR1)
  [in5] -> M035/3(T1)
  [in6] -> M035/4(EB1)
  [in7] -> M035/5(CT2)
  [in10] -> M035/6(MR2)
  [in11] -> M035/7(T2)
  [in12] -> M035/8(EB2)
  [in13] -> M035/9(CT3)
  [in14] -> M035/10(F3)
  [in15] -> M035/11(E3)
  [in17] -> M035/12(T3)
  [in18] -> M035/13(EB3)
  M035/1(LL1) -> Eval34/1(In1)
  M035/2(LL2) -> Eval34/2(In2)
  M035/3(LL3) -> Eval34/3(In3)
  Eval34/1(Out1) -> To Workspace34/1
  [in1] -> M046/1(CT1)
  [in4] -> M046/2(MR1)
  [in5] -> M046/3(T1)
  [in6] -> M046/4(EB1)
  [in7] -> M046/5(CT2)
  [in10] -> M046/6(MR2)
  [in11] -> M046/7(T2)
  [in12] -> M046/8(EB2)
  [in13] -> M046/9(CT3)
  [in14] -> M046/10(F3)
  [in15] -> M046/11(E3)
  [in17] -> M046/12(T3)
  [in18] -> M046/13(EB3)
  M046/1(LL1) -> Eval45/1(In1)
  M046/2(LL2) -> Eval45/2(In2)
  M046/3(LL3) -> Eval45/3(In3)
  Eval45/1(Out1) -> To Workspace45/1
  [in1] -> M047/1(CT1)
  [in4] -> M047/2(MR1)
  [in5] -> M047/3(T1)
  [in6] -> M047/4(EB1)
  [in7] -> M047/5(CT2)
  [in10] -> M047/6(MR2)
  [in11] -> M047/7(T2)
  [in12] -> M047/8(EB2)
  [in13] -> M047/9(CT3)
  [in14] -> M047/10(F3)
  [in15] -> M047/11(E3)
  [in17] -> M047/12(T3)
  [in18] -> M047/13(EB3)
  M047/1(LL1) -> Eval46/1(In1)
  M047/2(LL2) -> Eval46/2(In2)
  M047/3(LL3) -> Eval46/3(In3)
  Eval46/1(Out1) -> To Workspace46/1
  [in1] -> M048/1(CT1)
  [in4] -> M048/2(MR1)
  [in5] -> M048/3(T1)
  [in6] -> M048/4(EB1)
  [in7] -> M048/5(CT2)
  [in10] -> M048/6(MR2)
  [in11] -> M048/7(T2)
  [in12] -> M048/8(EB2)
  [in13] -> M048/9(CT3)
  [in14] -> M048/10(F3)
  [in15] -> M048/11(E3)
  [in17] -> M048/12(T3)
  [in18] -> M048/13(EB3)
  M048/1(LL1) -> Eval47/1(In1)
  M048/2(LL2) -> Eval47/2(In2)
  M048/3(LL3) -> Eval47/3(In3)
  Eval47/1(Out1) -> To Workspace47/1
  [in1] -> M049/1(CT1)
  [in4] -> M049/2(MR1)
  [in5] -> M049/3(T1)
  [in6] -> M049/4(EB1)
  [in7] -> M049/5(CT2)
  [in10] -> M049/6(MR2)
  [in11] -> M049/7(T2)
  [in12] -> M049/8(EB2)
  [in13] -> M049/9(CT3)
  [in14] -> M049/10(F3)
  [in15] -> M049/11(E3)
  [in17] -> M049/12(T3)
  [in18] -> M049/13(EB3)
  M049/1(LL1) -> Eval48/1(In1)
  M049/2(LL2) -> Eval48/2(In2)
  M049/3(LL3) -> Eval48/3(In3)
  Eval48/1(Out1) -> To Workspace48/1
  [in1] -> M050/1(CT1)
  [in4] -> M050/2(MR1)
  [in5] -> M050/3(T1)
  [in6] -> M050/4(EB1)
  [in7] -> M050/5(CT2)
  [in10] -> M050/6(MR2)
  [in11] -> M050/7(T2)
  [in12] -> M050/8(EB2)
  [in13] -> M050/9(CT3)
  [in14] -> M050/10(F3)
  [in15] -> M050/11(E3)
  [in17] -> M050/12(T3)
  [in18] -> M050/13(EB3)
  M050/1(LL1) -> Eval49/1(In1)
  M050/2(LL2) -> Eval49/2(In2)
  M050/3(LL3) -> Eval49/3(In3)
  Eval49/1(Out1) -> To Workspace49/1
  [in1] -> M051/1(CT1)
  [in4] -> M051/2(MR1)
  [in5] -> M051/3(T1)
  [in6] -> M051/4(EB1)
  [in7] -> M051/5(CT2)
  [in10] -> M051/6(MR2)
  [in11] -> M051/7(T2)
  [in12] -> M051/8(EB2)
  [in13] -> M051/9(CT3)
  [in14] -> M051/10(F3)
  [in15] -> M051/11(E3)
  [in17] -> M051/12(T3)
  [in18] -> M051/13(EB3)
  M051/1(LL1) -> Eval50/1(In1)
  M051/2(LL2) -> Eval50/2(In2)
  M051/3(LL3) -> Eval50/3(In3)
  Eval50/1(Out1) -> To Workspace50/1
  [in1] -> M052/1(CT1)
  [in4] -> M052/2(MR1)
  [in5] -> M052/3(T1)
  [in6] -> M052/4(EB1)
  [in7] -> M052/5(CT2)
  [in10] -> M052/6(MR2)
  [in11] -> M052/7(T2)
  [in12] -> M052/8(EB2)
  [in13] -> M052/9(CT3)
  [in14] -> M052/10(F3)
  [in15] -> M052/11(E3)
  [in17] -> M052/12(T3)
  [in18] -> M052/13(EB3)
  M052/1(LL1) -> Eval51/1(In1)
  M052/2(LL2) -> Eval51/2(In2)
  M052/3(LL3) -> Eval51/3(In3)
  Eval51/1(Out1) -> To Workspace51/1
  [in1] -> M053/1(CT1)
  [in4] -> M053/2(MR1)
  [in5] -> M053/3(T1)
  [in6] -> M053/4(EB1)
  [in7] -> M053/5(CT2)
  [in10] -> M053/6(MR2)
  [in11] -> M053/7(T2)
  [in12] -> M053/8(EB2)
  [in13] -> M053/9(CT3)
  [in14] -> M053/10(F3)
  [in15] -> M053/11(E3)
  [in17] -> M053/12(T3)
  [in18] -> M053/13(EB3)
  M053/1(LL1) -> Eval52/1(In1)
  M053/2(LL2) -> Eval52/2(In2)
  M053/3(LL3) -> Eval52/3(In3)
  Eval52/1(Out1) -> To Workspace52/1
  [in1] -> M054/1(CT1)
  [in4] -> M054/2(MR1)
  [in5] -> M054/3(T1)
  [in6] -> M054/4(EB1)
  [in7] -> M054/5(CT2)
  [in10] -> M054/6(MR2)
  [in11] -> M054/7(T2)
  [in12] -> M054/8(EB2)
  [in13] -> M054/9(CT3)
  [in14] -> M054/10(F3)
  [in15] -> M054/11(E3)
  [in17] -> M054/12(T3)
  [in18] -> M054/13(EB3)
  M054/1(LL1) -> Eval53/1(In1)
  M054/2(LL2) -> Eval53/2(In2)
  M054/3(LL3) -> Eval53/3(In3)
  Eval53/1(Out1) -> To Workspace53/1
  [in1] -> M055/1(CT1)
  [in4] -> M055/2(MR1)
  [in5] -> M055/3(T1)
  [in6] -> M055/4(EB1)
  [in7] -> M055/5(CT2)
  [in10] -> M055/6(MR2)
  [in11] -> M055/7(T2)
  [in12] -> M055/8(EB2)
  [in13] -> M055/9(CT3)
  [in14] -> M055/10(F3)
  [in15] -> M055/11(E3)
  [in17] -> M055/12(T3)
  [in18] -> M055/13(EB3)
  M055/1(LL1) -> Eval54/1(In1)
  M055/2(LL2) -> Eval54/2(In2)
  M055/3(LL3) -> Eval54/3(In3)
  Eval54/1(Out1) -> To Workspace54/1
  [in1] -> M056/1(CT1)
  [in4] -> M056/2(MR1)
  [in5] -> M056/3(T1)
  [in6] -> M056/4(EB1)
  [in7] -> M056/5(CT2)
  [in10] -> M056/6(MR2)
  [in11] -> M056/7(T2)
  [in12] -> M056/8(EB2)
  [in13] -> M056/9(CT3)
  [in14] -> M056/10(F3)
  [in15] -> M056/11(E3)
  [in17] -> M056/12(T3)
  [in18] -> M056/13(EB3)
  M056/1(LL1) -> Eval55/1(In1)
  M056/2(LL2) -> Eval55/2(In2)
  M056/3(LL3) -> Eval55/3(In3)
  Eval55/1(Out1) -> To Workspace55/1
  [in1] -> M058/1(CT1)
  [in4] -> M058/2(MR1)
  [in5] -> M058/3(T1)
  [in6] -> M058/4(EB1)
  [in7] -> M058/5(CT2)
  [in10] -> M058/6(MR2)
  [in11] -> M058/7(T2)
  [in12] -> M058/8(EB2)
  [in13] -> M058/9(CT3)
  [in14] -> M058/10(F3)
  [in15] -> M058/11(E3)
  [in17] -> M058/12(T3)
  [in18] -> M058/13(EB3)
  M058/1(LL1) -> Eval57/1(In1)
  M058/2(LL2) -> Eval57/2(In2)
  M058/3(LL3) -> Eval57/3(In3)
  Eval57/1(Out1) -> To Workspace57/1
  [in1] -> M059/1(CT1)
  [in4] -> M059/2(MR1)
  [in5] -> M059/3(T1)
  [in6] -> M059/4(EB1)
  [in7] -> M059/5(CT2)
  [in10] -> M059/6(MR2)
  [in11] -> M059/7(T2)
  [in12] -> M059/8(EB2)
  [in13] -> M059/9(CT3)
  [in14] -> M059/10(F3)
  [in15] -> M059/11(E3)
  [in17] -> M059/12(T3)
  [in18] -> M059/13(EB3)
  M059/1(LL1) -> Eval58/1(In1)
  M059/2(LL2) -> Eval58/2(In2)
  M059/3(LL3) -> Eval58/3(In3)
  Eval58/1(Out1) -> To Workspace58/1
  [in1] -> M060/1(CT1)
  [in4] -> M060/2(MR1)
  [in5] -> M060/3(T1)
  [in6] -> M060/4(EB1)
  [in7] -> M060/5(CT2)
  [in10] -> M060/6(MR2)
  [in11] -> M060/7(T2)
  [in12] -> M060/8(EB2)
  [in13] -> M060/9(CT3)
  [in14] -> M060/10(F3)
  [in15] -> M060/11(E3)
  [in17] -> M060/12(T3)
  [in18] -> M060/13(EB3)
  M060/1(LL1) -> Eval59/1(In1)
  M060/2(LL2) -> Eval59/2(In2)
  M060/3(LL3) -> Eval59/3(In3)
  Eval59/1(Out1) -> To Workspace59/1
  [in1] -> M061/1(CT1)
  [in4] -> M061/2(MR1)
  [in5] -> M061/3(T1)
  [in6] -> M061/4(EB1)
  [in7] -> M061/5(CT2)
  [in10] -> M061/6(MR2)
  [in11] -> M061/7(T2)
  [in12] -> M061/8(EB2)
  [in13] -> M061/9(CT3)
  [in14] -> M061/10(F3)
  [in15] -> M061/11(E3)
  [in17] -> M061/12(T3)
  [in18] -> M061/13(EB3)
  M061/1(LL1) -> Eval60/1(In1)
  M061/2(LL2) -> Eval60/2(In2)
  M061/3(LL3) -> Eval60/3(In3)
  Eval60/1(Out1) -> To Workspace60/1
  [in1] -> M062/1(CT1)
  [in4] -> M062/2(MR1)
  [in5] -> M062/3(T1)
  [in6] -> M062/4(EB1)
  [in7] -> M062/5(CT2)
  [in10] -> M062/6(MR2)
  [in11] -> M062/7(T2)
  [in12] -> M062/8(EB2)
  [in13] -> M062/9(CT3)
  [in14] -> M062/10(F3)
  [in15] -> M062/11(E3)
  [in17] -> M062/12(T3)
  [in18] -> M062/13(EB3)
  M062/1(LL1) -> Eval61/1(In1)
  M062/2(LL2) -> Eval61/2(In2)
  M062/3(LL3) -> Eval61/3(In3)
  Eval61/1(Out1) -> To Workspace61/1
  [in1] -> M063/1(CT1)
  [in4] -> M063/2(MR1)
  [in5] -> M063/3(T1)
  [in6] -> M063/4(EB1)
  [in7] -> M063/5(CT2)
  [in10] -> M063/6(MR2)
  [in11] -> M063/7(T2)
  [in12] -> M063/8(EB2)
  [in13] -> M063/9(CT3)
  [in14] -> M063/10(F3)
  [in15] -> M063/11(E3)
  [in17] -> M063/12(T3)
  [in18] -> M063/13(EB3)
  M063/1(LL1) -> Eval62/1(In1)
  M063/2(LL2) -> Eval62/2(In2)
  M063/3(LL3) -> Eval62/3(In3)
  Eval62/1(Out1) -> To Workspace62/1
  [in1] -> M064/1(CT1)
  [in4] -> M064/2(MR1)
  [in5] -> M064/3(T1)
  [in6] -> M064/4(EB1)
  [in7] -> M064/5(CT2)
  [in10] -> M064/6(MR2)
  [in11] -> M064/7(T2)
  [in12] -> M064/8(EB2)
  [in13] -> M064/9(CT3)
  [in14] -> M064/10(F3)
  [in15] -> M064/11(E3)
  [in17] -> M064/12(T3)
  [in18] -> M064/13(EB3)
  M064/1(LL1) -> Eval63/1(In1)
  M064/2(LL2) -> Eval63/2(In2)
  M064/3(LL3) -> Eval63/3(In3)
  Eval63/1(Out1) -> To Workspace63/1
  [in1] -> M065/1(CT1)
  [in4] -> M065/2(MR1)
  [in5] -> M065/3(T1)
  [in6] -> M065/4(EB1)
  [in7] -> M065/5(CT2)
  [in10] -> M065/6(MR2)
  [in11] -> M065/7(T2)
  [in12] -> M065/8(EB2)
  [in13] -> M065/9(CT3)
  [in14] -> M065/10(F3)
  [in15] -> M065/11(E3)
  [in17] -> M065/12(T3)
  [in18] -> M065/13(EB3)
  M065/1(LL1) -> Eval64/1(In1)
  M065/2(LL2) -> Eval64/2(In2)
  M065/3(LL3) -> Eval64/3(In3)
  Eval64/1(Out1) -> To Workspace64/1
  [in1] -> M066/1(CT1)
  [in4] -> M066/2(MR1)
  [in5] -> M066/3(T1)
  [in6] -> M066/4(EB1)
  [in7] -> M066/5(CT2)
  [in10] -> M066/6(MR2)
  [in11] -> M066/7(T2)
  [in12] -> M066/8(EB2)
  [in13] -> M066/9(CT3)
  [in14] -> M066/10(F3)
  [in15] -> M066/11(E3)
  [in17] -> M066/12(T3)
  [in18] -> M066/13(EB3)
  M066/1(LL1) -> Eval65/1(In1)
  M066/2(LL2) -> Eval65/2(In2)
  M066/3(LL3) -> Eval65/3(In3)
  Eval65/1(Out1) -> To Workspace65/1
  [in1] -> M067/1(CT1)
  [in4] -> M067/2(MR1)
  [in5] -> M067/3(T1)
  [in6] -> M067/4(EB1)
  [in7] -> M067/5(CT2)
  [in10] -> M067/6(MR2)
  [in11] -> M067/7(T2)
  [in12] -> M067/8(EB2)
  [in13] -> M067/9(CT3)
  [in14] -> M067/10(F3)
  [in15] -> M067/11(E3)
  [in17] -> M067/12(T3)
  [in18] -> M067/13(EB3)
  M067/1(LL1) -> Eval66/1(In1)
  M067/2(LL2) -> Eval66/2(In2)
  M067/3(LL3) -> Eval66/3(In3)
  Eval66/1(Out1) -> To Workspace66/1
  [in1] -> M068/1(CT1)
  [in4] -> M068/2(MR1)
  [in5] -> M068/3(T1)
  [in6] -> M068/4(EB1)
  [in7] -> M068/5(CT2)
  [in10] -> M068/6(MR2)
  [in11] -> M068/7(T2)
  [in12] -> M068/8(EB2)
  [in13] -> M068/9(CT3)
  [in14] -> M068/10(F3)
  [in15] -> M068/11(E3)
  [in17] -> M068/12(T3)
  [in18] -> M068/13(EB3)
  M068/1(LL1) -> Eval67/1(In1)
  M068/2(LL2) -> Eval67/2(In2)
  M068/3(LL3) -> Eval67/3(In3)
  Eval67/1(Out1) -> To Workspace67/1
  [in1] -> M069/1(CT1)
  [in4] -> M069/2(MR1)
  [in5] -> M069/3(T1)
  [in6] -> M069/4(EB1)
  [in7] -> M069/5(CT2)
  [in10] -> M069/6(MR2)
  [in11] -> M069/7(T2)
  [in12] -> M069/8(EB2)
  [in13] -> M069/9(CT3)
  [in14] -> M069/10(F3)
  [in15] -> M069/11(E3)
  [in17] -> M069/12(T3)
  [in18] -> M069/13(EB3)
  M069/1(LL1) -> Eval68/1(In1)
  M069/2(LL2) -> Eval68/2(In2)
  M069/3(LL3) -> Eval68/3(In3)
  Eval68/1(Out1) -> To Workspace68/1
  [in1] -> M070/1(CT1)
  [in4] -> M070/2(MR1)
  [in5] -> M070/3(T1)
  [in6] -> M070/4(EB1)
  [in7] -> M070/5(CT2)
  [in10] -> M070/6(MR2)
  [in11] -> M070/7(T2)
  [in12] -> M070/8(EB2)
  [in13] -> M070/9(CT3)
  [in14] -> M070/10(F3)
  [in15] -> M070/11(E3)
  [in17] -> M070/12(T3)
  [in18] -> M070/13(EB3)
  M070/1(LL1) -> Eval69/1(In1)
  M070/2(LL2) -> Eval69/2(In2)
  M070/3(LL3) -> Eval69/3(In3)
  Eval69/1(Out1) -> To Workspace69/1
  [in1] -> M071/1(CT1)
  [in4] -> M071/2(MR1)
  [in5] -> M071/3(T1)
  [in6] -> M071/4(EB1)
  [in7] -> M071/5(CT2)
  [in10] -> M071/6(MR2)
  [in11] -> M071/7(T2)
  [in12] -> M071/8(EB2)
  [in13] -> M071/9(CT3)
  [in14] -> M071/10(F3)
  [in15] -> M071/11(E3)
  [in17] -> M071/12(T3)
  [in18] -> M071/13(EB3)
  M071/1(LL1) -> Eval70/1(In1)
  M071/2(LL2) -> Eval70/2(In2)
  M071/3(LL3) -> Eval70/3(In3)
  Eval70/1(Out1) -> To Workspace70/1
  [in1] -> M072/1(CT1)
  [in4] -> M072/2(MR1)
  [in5] -> M072/3(T1)
  [in6] -> M072/4(EB1)
  [in7] -> M072/5(CT2)
  [in10] -> M072/6(MR2)
  [in11] -> M072/7(T2)
  [in12] -> M072/8(EB2)
  [in13] -> M072/9(CT3)
  [in14] -> M072/10(F3)
  [in15] -> M072/11(E3)
  [in17] -> M072/12(T3)
  [in18] -> M072/13(EB3)
  M072/1(LL1) -> Eval71/1(In1)
  M072/2(LL2) -> Eval71/2(In2)
  M072/3(LL3) -> Eval71/3(In3)
  Eval71/1(Out1) -> To Workspace71/1
  [in1] -> M073/1(CT1)
  [in4] -> M073/2(MR1)
  [in5] -> M073/3(T1)
  [in6] -> M073/4(EB1)
  [in7] -> M073/5(CT2)
  [in10] -> M073/6(MR2)
  [in11] -> M073/7(T2)
  [in12] -> M073/8(EB2)
  [in13] -> M073/9(CT3)
  [in14] -> M073/10(F3)
  [in15] -> M073/11(E3)
  [in17] -> M073/12(T3)
  [in18] -> M073/13(EB3)
  M073/1(LL1) -> Eval72/1(In1)
  M073/2(LL2) -> Eval72/2(In2)
  M073/3(LL3) -> Eval72/3(In3)
  Eval72/1(Out1) -> To Workspace72/1
  [in1] -> M074/1(CT1)
  [in4] -> M074/2(MR1)
  [in5] -> M074/3(T1)
  [in6] -> M074/4(EB1)
  [in7] -> M074/5(CT2)
  [in10] -> M074/6(MR2)
  [in11] -> M074/7(T2)
  [in12] -> M074/8(EB2)
  [in13] -> M074/9(CT3)
  [in14] -> M074/10(F3)
  [in15] -> M074/11(E3)
  [in17] -> M074/12(T3)
  [in18] -> M074/13(EB3)
  M074/1(LL1) -> Eval73/1(In1)
  M074/2(LL2) -> Eval73/2(In2)
  M074/3(LL3) -> Eval73/3(In3)
  Eval73/1(Out1) -> To Workspace73/1
  [in1] -> M075/1(CT1)
  [in4] -> M075/2(MR1)
  [in5] -> M075/3(T1)
  [in6] -> M075/4(EB1)
  [in7] -> M075/5(CT2)
  [in10] -> M075/6(MR2)
  [in11] -> M075/7(T2)
  [in12] -> M075/8(EB2)
  [in13] -> M075/9(CT3)
  [in14] -> M075/10(F3)
  [in15] -> M075/11(E3)
  [in17] -> M075/12(T3)
  [in18] -> M075/13(EB3)
  M075/1(LL1) -> Eval74/1(In1)
  M075/2(LL2) -> Eval74/2(In2)
  M075/3(LL3) -> Eval74/3(In3)
  Eval74/1(Out1) -> To Workspace74/1
  [in1] -> M076/1(CT1)
  [in4] -> M076/2(MR1)
  [in5] -> M076/3(T1)
  [in6] -> M076/4(EB1)
  [in7] -> M076/5(CT2)
  [in10] -> M076/6(MR2)
  [in11] -> M076/7(T2)
  [in12] -> M076/8(EB2)
  [in13] -> M076/9(CT3)
  [in14] -> M076/10(F3)
  [in15] -> M076/11(E3)
  [in17] -> M076/12(T3)
  [in18] -> M076/13(EB3)
  M076/1(LL1) -> Eval75/1(In1)
  M076/2(LL2) -> Eval75/2(In2)
  M076/3(LL3) -> Eval75/3(In3)
  Eval75/1(Out1) -> To Workspace75/1
  [in1] -> M077/1(CT1)
  [in4] -> M077/2(MR1)
  [in5] -> M077/3(T1)
  [in6] -> M077/4(EB1)
  [in7] -> M077/5(CT2)
  [in10] -> M077/6(MR2)
  [in11] -> M077/7(T2)
  [in12] -> M077/8(EB2)
  [in13] -> M077/9(CT3)
  [in14] -> M077/10(F3)
  [in15] -> M077/11(E3)
  [in17] -> M077/12(T3)
  [in18] -> M077/13(EB3)
  M077/1(LL1) -> Eval76/1(In1)
  M077/2(LL2) -> Eval76/2(In2)
  M077/3(LL3) -> Eval76/3(In3)
  Eval76/1(Out1) -> To Workspace76/1
  [in1] -> M078/1(CT1)
  [in4] -> M078/2(MR1)
  [in5] -> M078/3(T1)
  [in6] -> M078/4(EB1)
  [in7] -> M078/5(CT2)
  [in10] -> M078/6(MR2)
  [in11] -> M078/7(T2)
  [in12] -> M078/8(EB2)
  [in13] -> M078/9(CT3)
  [in14] -> M078/10(F3)
  [in15] -> M078/11(E3)
  [in17] -> M078/12(T3)
  [in18] -> M078/13(EB3)
  M078/1(LL1) -> Eval77/1(In1)
  M078/2(LL2) -> Eval77/2(In2)
  M078/3(LL3) -> Eval77/3(In3)
  Eval77/1(Out1) -> To Workspace77/1
  [in1] -> M079/1(CT1)
  [in4] -> M079/2(MR1)
  [in5] -> M079/3(T1)
  [in6] -> M079/4(EB1)
  [in7] -> M079/5(CT2)
  [in10] -> M079/6(MR2)
  [in11] -> M079/7(T2)
  [in12] -> M079/8(EB2)
  [in13] -> M079/9(CT3)
  [in14] -> M079/10(F3)
  [in15] -> M079/11(E3)
  [in17] -> M079/12(T3)
  [in18] -> M079/13(EB3)
  M079/1(LL1) -> Eval78/1(In1)
  M079/2(LL2) -> Eval78/2(In2)
  M079/3(LL3) -> Eval78/3(In3)
  Eval78/1(Out1) -> To Workspace78/1
  [in1] -> M080/1(CT1)
  [in4] -> M080/2(MR1)
  [in5] -> M080/3(T1)
  [in6] -> M080/4(EB1)
  [in7] -> M080/5(CT2)
  [in10] -> M080/6(MR2)
  [in11] -> M080/7(T2)
  [in12] -> M080/8(EB2)
  [in13] -> M080/9(CT3)
  [in14] -> M080/10(F3)
  [in15] -> M080/11(E3)
  [in17] -> M080/12(T3)
  [in18] -> M080/13(EB3)
  M080/1(LL1) -> Eval79/1(In1)
  M080/2(LL2) -> Eval79/2(In2)
  M080/3(LL3) -> Eval79/3(In3)
  Eval79/1(Out1) -> To Workspace79/1
  [in1] -> M081/1(CT1)
  [in4] -> M081/2(MR1)
  [in5] -> M081/3(T1)
  [in6] -> M081/4(EB1)
  [in7] -> M081/5(CT2)
  [in10] -> M081/6(MR2)
  [in11] -> M081/7(T2)
  [in12] -> M081/8(EB2)
  [in13] -> M081/9(CT3)
  [in14] -> M081/10(F3)
  [in15] -> M081/11(E3)
  [in17] -> M081/12(T3)
  [in18] -> M081/13(EB3)
  M081/1(LL1) -> Eval80/1(In1)
  M081/2(LL2) -> Eval80/2(In2)
  M081/3(LL3) -> Eval80/3(In3)
  Eval80/1(Out1) -> To Workspace80/1
  [in1] -> M082/1(CT1)
  [in4] -> M082/2(MR1)
  [in5] -> M082/3(T1)
  [in6] -> M082/4(EB1)
  [in7] -> M082/5(CT2)
  [in10] -> M082/6(MR2)
  [in11] -> M082/7(T2)
  [in12] -> M082/8(EB2)
  [in13] -> M082/9(CT3)
  [in14] -> M082/10(F3)
  [in15] -> M082/11(E3)
  [in17] -> M082/12(T3)
  [in18] -> M082/13(EB3)
  M082/1(LL1) -> Eval81/1(In1)
  M082/2(LL2) -> Eval81/2(In2)
  M082/3(LL3) -> Eval81/3(In3)
  Eval81/1(Out1) -> To Workspace81/1
  [in1] -> M083/1(CT1)
  [in4] -> M083/2(MR1)
  [in5] -> M083/3(T1)
  [in6] -> M083/4(EB1)
  [in7] -> M083/5(CT2)
  [in10] -> M083/6(MR2)
  [in11] -> M083/7(T2)
  [in12] -> M083/8(EB2)
  [in13] -> M083/9(CT3)
  [in14] -> M083/10(F3)
  [in15] -> M083/11(E3)
  [in17] -> M083/12(T3)
  [in18] -> M083/13(EB3)
  M083/1(LL1) -> Eval82/1(In1)
  M083/2(LL2) -> Eval82/2(In2)
  M083/3(LL3) -> Eval82/3(In3)
  Eval82/1(Out1) -> To Workspace82/1
  [in1] -> M087/1(CT1)
  [in4] -> M087/2(MR1)
  [in5] -> M087/3(T1)
  [in6] -> M087/4(EB1)
  [in7] -> M087/5(CT2)
  [in10] -> M087/6(MR2)
  [in11] -> M087/7(T2)
  [in12] -> M087/8(EB2)
  [in13] -> M087/9(CT3)
  [in14] -> M087/10(F3)
  [in15] -> M087/11(E3)
  [in17] -> M087/12(T3)
  [in18] -> M087/13(EB3)
  M087/1(LL1) -> Eval86/1(In1)
  M087/2(LL2) -> Eval86/2(In2)
  M087/3(LL3) -> Eval86/3(In3)
  Eval86/1(Out1) -> To Workspace86/1
  [in1] -> M088/1(CT1)
  [in4] -> M088/2(MR1)
  [in5] -> M088/3(T1)
  [in6] -> M088/4(EB1)
  [in7] -> M088/5(CT2)
  [in10] -> M088/6(MR2)
  [in11] -> M088/7(T2)
  [in12] -> M088/8(EB2)
  [in13] -> M088/9(CT3)
  [in14] -> M088/10(F3)
  [in15] -> M088/11(E3)
  [in17] -> M088/12(T3)
  [in18] -> M088/13(EB3)
  M088/1(LL1) -> Eval87/1(In1)
  M088/2(LL2) -> Eval87/2(In2)
  M088/3(LL3) -> Eval87/3(In3)
  Eval87/1(Out1) -> To Workspace87/1
  [in1] -> M089/1(CT1)
  [in4] -> M089/2(MR1)
  [in5] -> M089/3(T1)
  [in6] -> M089/4(EB1)
  [in7] -> M089/5(CT2)
  [in10] -> M089/6(MR2)
  [in11] -> M089/7(T2)
  [in12] -> M089/8(EB2)
  [in13] -> M089/9(CT3)
  [in14] -> M089/10(F3)
  [in15] -> M089/11(E3)
  [in17] -> M089/12(T3)
  [in18] -> M089/13(EB3)
  M089/1(LL1) -> Eval88/1(In1)
  M089/2(LL2) -> Eval88/2(In2)
  M089/3(LL3) -> Eval88/3(In3)
  Eval88/1(Out1) -> To Workspace88/1
  [in1] -> M090/1(CT1)
  [in4] -> M090/2(MR1)
  [in5] -> M090/3(T1)
  [in6] -> M090/4(EB1)
  [in7] -> M090/5(CT2)
  [in10] -> M090/6(MR2)
  [in11] -> M090/7(T2)
  [in12] -> M090/8(EB2)
  [in13] -> M090/9(CT3)
  [in14] -> M090/10(F3)
  [in15] -> M090/11(E3)
  [in17] -> M090/12(T3)
  [in18] -> M090/13(EB3)
  M090/1(LL1) -> Eval89/1(In1)
  M090/2(LL2) -> Eval89/2(In2)
  M090/3(LL3) -> Eval89/3(In3)
  Eval89/1(Out1) -> To Workspace89/1
  [in1] -> M091/1(CT1)
  [in4] -> M091/2(MR1)
  [in5] -> M091/3(T1)
  [in6] -> M091/4(EB1)
  [in7] -> M091/5(CT2)
  [in10] -> M091/6(MR2)
  [in11] -> M091/7(T2)
  [in12] -> M091/8(EB2)
  [in13] -> M091/9(CT3)
  [in14] -> M091/10(F3)
  [in15] -> M091/11(E3)
  [in17] -> M091/12(T3)
  [in18] -> M091/13(EB3)
  M091/1(LL1) -> Eval90/1(In1)
  M091/2(LL2) -> Eval90/2(In2)
  M091/3(LL3) -> Eval90/3(In3)
  Eval90/1(Out1) -> To Workspace90/1
  [in1] -> M092/1(CT1)
  [in4] -> M092/2(MR1)
  [in5] -> M092/3(T1)
  [in6] -> M092/4(EB1)
  [in7] -> M092/5(CT2)
  [in10] -> M092/6(MR2)
  [in11] -> M092/7(T2)
  [in12] -> M092/8(EB2)
  [in13] -> M092/9(CT3)
  [in14] -> M092/10(F3)
  [in15] -> M092/11(E3)
  [in17] -> M092/12(T3)
  [in18] -> M092/13(EB3)
  M092/1(LL1) -> Eval91/1(In1)
  M092/2(LL2) -> Eval91/2(In2)
  M092/3(LL3) -> Eval91/3(In3)
  Eval91/1(Out1) -> To Workspace91/1
  [in1] -> M093/1(CT1)
  [in4] -> M093/2(MR1)
  [in5] -> M093/3(T1)
  [in6] -> M093/4(EB1)
  [in7] -> M093/5(CT2)
  [in10] -> M093/6(MR2)
  [in11] -> M093/7(T2)
  [in12] -> M093/8(EB2)
  [in13] -> M093/9(CT3)
  [in14] -> M093/10(F3)
  [in15] -> M093/11(E3)
  [in17] -> M093/12(T3)
  [in18] -> M093/13(EB3)
  M093/1(LL1) -> Eval92/1(In1)
  M093/2(LL2) -> Eval92/2(In2)
  M093/3(LL3) -> Eval92/3(In3)
  Eval92/1(Out1) -> To Workspace92/1
  [in1] -> M094/1(CT1)
  [in4] -> M094/2(MR1)
  [in5] -> M094/3(T1)
  [in6] -> M094/4(EB1)
  [in7] -> M094/5(CT2)
  [in10] -> M094/6(MR2)
  [in11] -> M094/7(T2)
  [in12] -> M094/8(EB2)
  [in13] -> M094/9(CT3)
  [in14] -> M094/10(F3)
  [in15] -> M094/11(E3)
  [in17] -> M094/12(T3)
  [in18] -> M094/13(EB3)
  M094/1(LL1) -> Eval93/1(In1)
  M094/2(LL2) -> Eval93/2(In2)
  M094/3(LL3) -> Eval93/3(In3)
  Eval93/1(Out1) -> To Workspace93/1
  [in1] -> M095/1(CT1)
  [in4] -> M095/2(MR1)
  [in5] -> M095/3(T1)
  [in6] -> M095/4(EB1)
  [in7] -> M095/5(CT2)
  [in10] -> M095/6(MR2)
  [in11] -> M095/7(T2)
  [in12] -> M095/8(EB2)
  [in13] -> M095/9(CT3)
  [in14] -> M095/10(F3)
  [in15] -> M095/11(E3)
  [in17] -> M095/12(T3)
  [in18] -> M095/13(EB3)
  M095/1(LL1) -> Eval94/1(In1)
  M095/2(LL2) -> Eval94/2(In2)
  M095/3(LL3) -> Eval94/3(In3)
  Eval94/1(Out1) -> To Workspace94/1
  [in1] -> M096/1(CT1)
  [in4] -> M096/2(MR1)
  [in5] -> M096/3(T1)
  [in6] -> M096/4(EB1)
  [in7] -> M096/5(CT2)
  [in10] -> M096/6(MR2)
  [in11] -> M096/7(T2)
  [in12] -> M096/8(EB2)
  [in13] -> M096/9(CT3)
  [in14] -> M096/10(F3)
  [in15] -> M096/11(E3)
  [in17] -> M096/12(T3)
  [in18] -> M096/13(EB3)
  M096/1(LL1) -> Eval95/1(In1)
  M096/2(LL2) -> Eval95/2(In2)
  M096/3(LL3) -> Eval95/3(In3)
  Eval95/1(Out1) -> To Workspace95/1
  [in1] -> M097/1(CT1)
  [in4] -> M097/2(MR1)
  [in5] -> M097/3(T1)
  [in6] -> M097/4(EB1)
  [in7] -> M097/5(CT2)
  [in10] -> M097/6(MR2)
  [in11] -> M097/7(T2)
  [in12] -> M097/8(EB2)
  [in13] -> M097/9(CT3)
  [in14] -> M097/10(F3)
  [in15] -> M097/11(E3)
  [in17] -> M097/12(T3)
  [in18] -> M097/13(EB3)
  M097/1(LL1) -> Eval96/1(In1)
  M097/2(LL2) -> Eval96/2(In2)
  M097/3(LL3) -> Eval96/3(In3)
  Eval96/1(Out1) -> To Workspace96/1
  [in1] -> M098/1(CT1)
  [in4] -> M098/2(MR1)
  [in5] -> M098/3(T1)
  [in6] -> M098/4(EB1)
  [in7] -> M098/5(CT2)
  [in10] -> M098/6(MR2)
  [in11] -> M098/7(T2)
  [in12] -> M098/8(EB2)
  [in13] -> M098/9(CT3)
  [in14] -> M098/10(F3)
  [in15] -> M098/11(E3)
  [in17] -> M098/12(T3)
  [in18] -> M098/13(EB3)
  M098/1(LL1) -> Eval97/1(In1)
  M098/2(LL2) -> Eval97/2(In2)
  M098/3(LL3) -> Eval97/3(In3)
  Eval97/1(Out1) -> To Workspace97/1
  [in1] -> M099/1(CT1)
  [in4] -> M099/2(MR1)
  [in5] -> M099/3(T1)
  [in6] -> M099/4(EB1)
  [in7] -> M099/5(CT2)
  [in10] -> M099/6(MR2)
  [in11] -> M099/7(T2)
  [in12] -> M099/8(EB2)
  [in13] -> M099/9(CT3)
  [in14] -> M099/10(F3)
  [in15] -> M099/11(E3)
  [in17] -> M099/12(T3)
  [in18] -> M099/13(EB3)
  M099/1(LL1) -> Eval98/1(In1)
  M099/2(LL2) -> Eval98/2(In2)
  M099/3(LL3) -> Eval98/3(In3)
  Eval98/1(Out1) -> To Workspace98/1
  [in1] -> M100/1(CT1)
  [in4] -> M100/2(MR1)
  [in5] -> M100/3(T1)
  [in6] -> M100/4(EB1)
  [in7] -> M100/5(CT2)
  [in10] -> M100/6(MR2)
  [in11] -> M100/7(T2)
  [in12] -> M100/8(EB2)
  [in13] -> M100/9(CT3)
  [in14] -> M100/10(F3)
  [in15] -> M100/11(E3)
  [in17] -> M100/12(T3)
  [in18] -> M100/13(EB3)
  M100/1(LL1) -> Eval99/1(In1)
  M100/2(LL2) -> Eval99/2(In2)
  M100/3(LL3) -> Eval99/3(In3)
  Eval99/1(Out1) -> To Workspace99/1
  [in1] -> M101/1(CT1)
  [in4] -> M101/2(MR1)
  [in5] -> M101/3(T1)
  [in6] -> M101/4(EB1)
  [in7] -> M101/5(CT2)
  [in10] -> M101/6(MR2)
  [in11] -> M101/7(T2)
  [in12] -> M101/8(EB2)
  [in13] -> M101/9(CT3)
  [in14] -> M101/10(F3)
  [in15] -> M101/11(E3)
  [in17] -> M101/12(T3)
  [in18] -> M101/13(EB3)
  M101/1(LL1) -> Eval100/1(In1)
  M101/2(LL2) -> Eval100/2(In2)
  M101/3(LL3) -> Eval100/3(In3)
  Eval100/1(Out1) -> To Workspace100/1
  [in1] -> M102/1(CT1)
  [in4] -> M102/2(MR1)
  [in5] -> M102/3(T1)
  [in6] -> M102/4(EB1)
  [in7] -> M102/5(CT2)
  [in10] -> M102/6(MR2)
  [in11] -> M102/7(T2)
  [in12] -> M102/8(EB2)
  [in13] -> M102/9(CT3)
  [in14] -> M102/10(F3)
  [in15] -> M102/11(E3)
  [in17] -> M102/12(T3)
  [in18] -> M102/13(EB3)
  M102/1(LL1) -> Eval101/1(In1)
  M102/2(LL2) -> Eval101/2(In2)
  M102/3(LL3) -> Eval101/3(In3)
  Eval101/1(Out1) -> To Workspace101/1
  [in1] -> M103/1(CT1)
  [in4] -> M103/2(MR1)
  [in5] -> M103/3(T1)
  [in6] -> M103/4(EB1)
  [in7] -> M103/5(CT2)
  [in10] -> M103/6(MR2)
  [in11] -> M103/7(T2)
  [in12] -> M103/8(EB2)
  [in13] -> M103/9(CT3)
  [in14] -> M103/10(F3)
  [in15] -> M103/11(E3)
  [in17] -> M103/12(T3)
  [in18] -> M103/13(EB3)
  M103/1(LL1) -> Eval102/1(In1)
  M103/2(LL2) -> Eval102/2(In2)
  M103/3(LL3) -> Eval102/3(In3)
  Eval102/1(Out1) -> To Workspace102/1
  [in1] -> M104/1(CT1)
  [in4] -> M104/2(MR1)
  [in5] -> M104/3(T1)
  [in6] -> M104/4(EB1)
  [in7] -> M104/5(CT2)
  [in10] -> M104/6(MR2)
  [in11] -> M104/7(T2)
  [in12] -> M104/8(EB2)
  [in13] -> M104/9(CT3)
  [in14] -> M104/10(F3)
  [in15] -> M104/11(E3)
  [in17] -> M104/12(T3)
  [in18] -> M104/13(EB3)
  M104/1(LL1) -> Eval103/1(In1)
  M104/2(LL2) -> Eval103/2(In2)
  M104/3(LL3) -> Eval103/3(In3)
  Eval103/1(Out1) -> To Workspace103/1
  [in1] -> M105/1(CT1)
  [in4] -> M105/2(MR1)
  [in5] -> M105/3(T1)
  [in6] -> M105/4(EB1)
  [in7] -> M105/5(CT2)
  [in10] -> M105/6(MR2)
  [in11] -> M105/7(T2)
  [in12] -> M105/8(EB2)
  [in13] -> M105/9(CT3)
  [in14] -> M105/10(F3)
  [in15] -> M105/11(E3)
  [in17] -> M105/12(T3)
  [in18] -> M105/13(EB3)
  M105/1(LL1) -> Eval104/1(In1)
  M105/2(LL2) -> Eval104/2(In2)
  M105/3(LL3) -> Eval104/3(In3)
  Eval104/1(Out1) -> To Workspace104/1
  [in1] -> M106/1(CT1)
  [in4] -> M106/2(MR1)
  [in5] -> M106/3(T1)
  [in6] -> M106/4(EB1)
  [in7] -> M106/5(CT2)
  [in10] -> M106/6(MR2)
  [in11] -> M106/7(T2)
  [in12] -> M106/8(EB2)
  [in13] -> M106/9(CT3)
  [in14] -> M106/10(F3)
  [in15] -> M106/11(E3)
  [in17] -> M106/12(T3)
  [in18] -> M106/13(EB3)
  M106/1(LL1) -> Eval105/1(In1)
  M106/2(LL2) -> Eval105/2(In2)
  M106/3(LL3) -> Eval105/3(In3)
  Eval105/1(Out1) -> To Workspace105/1
  [in1] -> M107/1(CT1)
  [in4] -> M107/2(MR1)
  [in5] -> M107/3(T1)
  [in6] -> M107/4(EB1)
  [in7] -> M107/5(CT2)
  [in10] -> M107/6(MR2)
  [in11] -> M107/7(T2)
  [in12] -> M107/8(EB2)
  [in13] -> M107/9(CT3)
  [in14] -> M107/10(F3)
  [in15] -> M107/11(E3)
  [in17] -> M107/12(T3)
  [in18] -> M107/13(EB3)
  M107/1(LL1) -> Eval106/1(In1)
  M107/2(LL2) -> Eval106/2(In2)
  M107/3(LL3) -> Eval106/3(In3)
  Eval106/1(Out1) -> To Workspace106/1
  [in1] -> M108/1(CT1)
  [in4] -> M108/2(MR1)
  [in5] -> M108/3(T1)
  [in6] -> M108/4(EB1)
  [in7] -> M108/5(CT2)
  [in10] -> M108/6(MR2)
  [in11] -> M108/7(T2)
  [in12] -> M108/8(EB2)
  [in13] -> M108/9(CT3)
  [in14] -> M108/10(F3)
  [in15] -> M108/11(E3)
  [in17] -> M108/12(T3)
  [in18] -> M108/13(EB3)
  M108/1(LL1) -> Eval107/1(In1)
  M108/2(LL2) -> Eval107/2(In2)
  M108/3(LL3) -> Eval107/3(In3)
  Eval107/1(Out1) -> To Workspace107/1
  [in1] -> M109/1(CT1)
  [in4] -> M109/2(MR1)
  [in5] -> M109/3(T1)
  [in6] -> M109/4(EB1)
  [in7] -> M109/5(CT2)
  [in10] -> M109/6(MR2)
  [in11] -> M109/7(T2)
  [in12] -> M109/8(EB2)
  [in13] -> M109/9(CT3)
  [in14] -> M109/10(F3)
  [in15] -> M109/11(E3)
  [in17] -> M109/12(T3)
  [in18] -> M109/13(EB3)
  M109/1(LL1) -> Eval108/1(In1)
  M109/2(LL2) -> Eval108/2(In2)
  M109/3(LL3) -> Eval108/3(In3)
  Eval108/1(Out1) -> To Workspace108/1
  [in1] -> M110/1(CT1)
  [in4] -> M110/2(MR1)
  [in5] -> M110/3(T1)
  [in6] -> M110/4(EB1)
  [in7] -> M110/5(CT2)
  [in10] -> M110/6(MR2)
  [in11] -> M110/7(T2)
  [in12] -> M110/8(EB2)
  [in13] -> M110/9(CT3)
  [in14] -> M110/10(F3)
  [in15] -> M110/11(E3)
  [in17] -> M110/12(T3)
  [in18] -> M110/13(EB3)
  M110/1(LL1) -> Eval109/1(In1)
  M110/2(LL2) -> Eval109/2(In2)
  M110/3(LL3) -> Eval109/3(In3)
  Eval109/1(Out1) -> To Workspace109/1
  [in1] -> M111/1(CT1)
  [in4] -> M111/2(MR1)
  [in5] -> M111/3(T1)
  [in6] -> M111/4(EB1)
  [in7] -> M111/5(CT2)
  [in10] -> M111/6(MR2)
  [in11] -> M111/7(T2)
  [in12] -> M111/8(EB2)
  [in13] -> M111/9(CT3)
  [in14] -> M111/10(F3)
  [in15] -> M111/11(E3)
  [in17] -> M111/12(T3)
  [in18] -> M111/13(EB3)
  M111/1(LL1) -> Eval110/1(In1)
  M111/2(LL2) -> Eval110/2(In2)
  M111/3(LL3) -> Eval110/3(In3)
  Eval110/1(Out1) -> To Workspace110/1
  [in1] -> M112/1(CT1)
  [in4] -> M112/2(MR1)
  [in5] -> M112/3(T1)
  [in6] -> M112/4(EB1)
  [in7] -> M112/5(CT2)
  [in10] -> M112/6(MR2)
  [in11] -> M112/7(T2)
  [in12] -> M112/8(EB2)
  [in13] -> M112/9(CT3)
  [in14] -> M112/10(F3)
  [in15] -> M112/11(E3)
  [in17] -> M112/12(T3)
  [in18] -> M112/13(EB3)
  M112/1(LL1) -> Eval111/1(In1)
  M112/2(LL2) -> Eval111/2(In2)
  M112/3(LL3) -> Eval111/3(In3)
  Eval111/1(Out1) -> To Workspace111/1
  [in1] -> M113/1(CT1)
  [in4] -> M113/2(MR1)
  [in5] -> M113/3(T1)
  [in6] -> M113/4(EB1)
  [in7] -> M113/5(CT2)
  [in10] -> M113/6(MR2)
  [in11] -> M113/7(T2)
  [in12] -> M113/8(EB2)
  [in13] -> M113/9(CT3)
  [in14] -> M113/10(F3)
  [in15] -> M113/11(E3)
  [in17] -> M113/12(T3)
  [in18] -> M113/13(EB3)
  M113/1(LL1) -> Eval112/1(In1)
  M113/2(LL2) -> Eval112/2(In2)
  M113/3(LL3) -> Eval112/3(In3)
  Eval112/1(Out1) -> To Workspace112/1
  [in1] -> M114/1(CT1)
  [in4] -> M114/2(MR1)
  [in5] -> M114/3(T1)
  [in6] -> M114/4(EB1)
  [in7] -> M114/5(CT2)
  [in10] -> M114/6(MR2)
  [in11] -> M114/7(T2)
  [in12] -> M114/8(EB2)
  [in13] -> M114/9(CT3)
  [in14] -> M114/10(F3)
  [in15] -> M114/11(E3)
  [in17] -> M114/12(T3)
  [in18] -> M114/13(EB3)
  M114/1(LL1) -> Eval113/1(In1)
  M114/2(LL2) -> Eval113/2(In2)
  M114/3(LL3) -> Eval113/3(In3)
  Eval113/1(Out1) -> To Workspace113/1
  [in1] -> M115/1(CT1)
  [in4] -> M115/2(MR1)
  [in5] -> M115/3(T1)
  [in6] -> M115/4(EB1)
  [in7] -> M115/5(CT2)
  [in10] -> M115/6(MR2)
  [in11] -> M115/7(T2)
  [in12] -> M115/8(EB2)
  [in13] -> M115/9(CT3)
  [in14] -> M115/10(F3)
  [in15] -> M115/11(E3)
  [in17] -> M115/12(T3)
  [in18] -> M115/13(EB3)
  M115/1(LL1) -> Eval114/1(In1)
  M115/2(LL2) -> Eval114/2(In2)
  M115/3(LL3) -> Eval114/3(In3)
  Eval114/1(Out1) -> To Workspace114/1
  [in1] -> M116/1(CT1)
  [in4] -> M116/2(MR1)
  [in5] -> M116/3(T1)
  [in6] -> M116/4(EB1)
  [in7] -> M116/5(CT2)
  [in10] -> M116/6(MR2)
  [in11] -> M116/7(T2)
  [in12] -> M116/8(EB2)
  [in13] -> M116/9(CT3)
  [in14] -> M116/10(F3)
  [in15] -> M116/11(E3)
  [in17] -> M116/12(T3)
  [in18] -> M116/13(EB3)
  M116/1(LL1) -> Eval115/1(In1)
  M116/2(LL2) -> Eval115/2(In2)
  M116/3(LL3) -> Eval115/3(In3)
  Eval115/1(Out1) -> To Workspace115/1
  [in1] -> M117/1(CT1)
  [in4] -> M117/2(MR1)
  [in5] -> M117/3(T1)
  [in6] -> M117/4(EB1)
  [in7] -> M117/5(CT2)
  [in10] -> M117/6(MR2)
  [in11] -> M117/7(T2)
  [in12] -> M117/8(EB2)
  [in13] -> M117/9(CT3)
  [in14] -> M117/10(F3)
  [in15] -> M117/11(E3)
  [in17] -> M117/12(T3)
  [in18] -> M117/13(EB3)
  M117/1(LL1) -> Eval116/1(In1)
  M117/2(LL2) -> Eval116/2(In2)
  M117/3(LL3) -> Eval116/3(In3)
  Eval116/1(Out1) -> To Workspace116/1
  [in1] -> M128/1(CT1)
  [in4] -> M128/2(MR1)
  [in5] -> M128/3(T1)
  [in6] -> M128/4(EB1)
  [in7] -> M128/5(CT2)
  [in10] -> M128/6(MR2)
  [in11] -> M128/7(T2)
  [in12] -> M128/8(EB2)
  [in13] -> M128/9(CT3)
  [in14] -> M128/10(F3)
  [in15] -> M128/11(E3)
  [in17] -> M128/12(T3)
  [in18] -> M128/13(EB3)
  M128/1(LL1) -> Eval127/1(In1)
  M128/2(LL2) -> Eval127/2(In2)
  M128/3(LL3) -> Eval127/3(In3)
  Eval127/1(Out1) -> To Workspace127/1
  [in1] -> M129/1(CT1)
  [in4] -> M129/2(MR1)
  [in5] -> M129/3(T1)
  [in6] -> M129/4(EB1)
  [in7] -> M129/5(CT2)
  [in10] -> M129/6(MR2)
  [in11] -> M129/7(T2)
  [in12] -> M129/8(EB2)
  [in13] -> M129/9(CT3)
  [in14] -> M129/10(F3)
  [in15] -> M129/11(E3)
  [in17] -> M129/12(T3)
  [in18] -> M129/13(EB3)
  M129/1(LL1) -> Eval128/1(In1)
  M129/2(LL2) -> Eval128/2(In2)
  M129/3(LL3) -> Eval128/3(In3)
  Eval128/1(Out1) -> To Workspace128/1
  [in1] -> M130/1(CT1)
  [in4] -> M130/2(MR1)
  [in5] -> M130/3(T1)
  [in6] -> M130/4(EB1)
  [in7] -> M130/5(CT2)
  [in10] -> M130/6(MR2)
  [in11] -> M130/7(T2)
  [in12] -> M130/8(EB2)
  [in13] -> M130/9(CT3)
  [in14] -> M130/10(F3)
  [in15] -> M130/11(E3)
  [in17] -> M130/12(T3)
  [in18] -> M130/13(EB3)
  M130/1(LL1) -> Eval129/1(In1)
  M130/2(LL2) -> Eval129/2(In2)
  M130/3(LL3) -> Eval129/3(In3)
  Eval129/1(Out1) -> To Workspace129/1
  [in1] -> M131/1(CT1)
  [in4] -> M131/2(MR1)
  [in5] -> M131/3(T1)
  [in6] -> M131/4(EB1)
  [in7] -> M131/5(CT2)
  [in10] -> M131/6(MR2)
  [in11] -> M131/7(T2)
  [in12] -> M131/8(EB2)
  [in13] -> M131/9(CT3)
  [in14] -> M131/10(F3)
  [in15] -> M131/11(E3)
  [in17] -> M131/12(T3)
  [in18] -> M131/13(EB3)
  M131/1(LL1) -> Eval130/1(In1)
  M131/2(LL2) -> Eval130/2(In2)
  M131/3(LL3) -> Eval130/3(In3)
  Eval130/1(Out1) -> To Workspace130/1
  [in1] -> M132/1(CT1)
  [in4] -> M132/2(MR1)
  [in5] -> M132/3(T1)
  [in6] -> M132/4(EB1)
  [in7] -> M132/5(CT2)
  [in10] -> M132/6(MR2)
  [in11] -> M132/7(T2)
  [in12] -> M132/8(EB2)
  [in13] -> M132/9(CT3)
  [in14] -> M132/10(F3)
  [in15] -> M132/11(E3)
  [in17] -> M132/12(T3)
  [in18] -> M132/13(EB3)
  M132/1(LL1) -> Eval131/1(In1)
  M132/2(LL2) -> Eval131/2(In2)
  M132/3(LL3) -> Eval131/3(In3)
  Eval131/1(Out1) -> To Workspace131/1
  [in1] -> M133/1(CT1)
  [in4] -> M133/2(MR1)
  [in5] -> M133/3(T1)
  [in6] -> M133/4(EB1)
  [in7] -> M133/5(CT2)
  [in10] -> M133/6(MR2)
  [in11] -> M133/7(T2)
  [in12] -> M133/8(EB2)
  [in13] -> M133/9(CT3)
  [in14] -> M133/10(F3)
  [in15] -> M133/11(E3)
  [in17] -> M133/12(T3)
  [in18] -> M133/13(EB3)
  M133/1(LL1) -> Eval132/1(In1)
  M133/2(LL2) -> Eval132/2(In2)
  M133/3(LL3) -> Eval132/3(In3)
  Eval132/1(Out1) -> To Workspace132/1
  [in1] -> M134/1(CT1)
  [in4] -> M134/2(MR1)
  [in5] -> M134/3(T1)
  [in6] -> M134/4(EB1)
  [in7] -> M134/5(CT2)
  [in10] -> M134/6(MR2)
  [in11] -> M134/7(T2)
  [in12] -> M134/8(EB2)
  [in13] -> M134/9(CT3)
  [in14] -> M134/10(F3)
  [in15] -> M134/11(E3)
  [in17] -> M134/12(T3)
  [in18] -> M134/13(EB3)
  M134/1(LL1) -> Eval133/1(In1)
  M134/2(LL2) -> Eval133/2(In2)
  M134/3(LL3) -> Eval133/3(In3)
  Eval133/1(Out1) -> To Workspace133/1
  [in1] -> M135/1(CT1)
  [in4] -> M135/2(MR1)
  [in5] -> M135/3(T1)
  [in6] -> M135/4(EB1)
  [in7] -> M135/5(CT2)
  [in10] -> M135/6(MR2)
  [in11] -> M135/7(T2)
  [in12] -> M135/8(EB2)
  [in13] -> M135/9(CT3)
  [in14] -> M135/10(F3)
  [in15] -> M135/11(E3)
  [in17] -> M135/12(T3)
  [in18] -> M135/13(EB3)
  M135/1(LL1) -> Eval134/1(In1)
  M135/2(LL2) -> Eval134/2(In2)
  M135/3(LL3) -> Eval134/3(In3)
  Eval134/1(Out1) -> To Workspace134/1
  [in1] -> M136/1(CT1)
  [in4] -> M136/2(MR1)
  [in5] -> M136/3(T1)
  [in6] -> M136/4(EB1)
  [in7] -> M136/5(CT2)
  [in10] -> M136/6(MR2)
  [in11] -> M136/7(T2)
  [in12] -> M136/8(EB2)
  [in13] -> M136/9(CT3)
  [in14] -> M136/10(F3)
  [in15] -> M136/11(E3)
  [in17] -> M136/12(T3)
  [in18] -> M136/13(EB3)
  M136/1(LL1) -> Eval135/1(In1)
  M136/2(LL2) -> Eval135/2(In2)
  M136/3(LL3) -> Eval135/3(In3)
  Eval135/1(Out1) -> To Workspace135/1
  [in1] -> M137/1(CT1)
  [in4] -> M137/2(MR1)
  [in5] -> M137/3(T1)
  [in6] -> M137/4(EB1)
  [in7] -> M137/5(CT2)
  [in10] -> M137/6(MR2)
  [in11] -> M137/7(T2)
  [in12] -> M137/8(EB2)
  [in13] -> M137/9(CT3)
  [in14] -> M137/10(F3)
  [in15] -> M137/11(E3)
  [in17] -> M137/12(T3)
  [in18] -> M137/13(EB3)
  M137/1(LL1) -> Eval136/1(In1)
  M137/2(LL2) -> Eval136/2(In2)
  M137/3(LL3) -> Eval136/3(In3)
  Eval136/1(Out1) -> To Workspace136/1
  [in1] -> M138/1(CT1)
  [in4] -> M138/2(MR1)
  [in5] -> M138/3(T1)
  [in6] -> M138/4(EB1)
  [in7] -> M138/5(CT2)
  [in10] -> M138/6(MR2)
  [in11] -> M138/7(T2)
  [in12] -> M138/8(EB2)
  [in13] -> M138/9(CT3)
  [in14] -> M138/10(F3)
  [in15] -> M138/11(E3)
  [in17] -> M138/12(T3)
  [in18] -> M138/13(EB3)
  M138/1(LL1) -> Eval137/1(In1)
  M138/2(LL2) -> Eval137/2(In2)
  M138/3(LL3) -> Eval137/3(In3)
  Eval137/1(Out1) -> To Workspace137/1
  [in1] -> M140/1(CT1)
  [in4] -> M140/2(MR1)
  [in5] -> M140/3(T1)
  [in6] -> M140/4(EB1)
  [in7] -> M140/5(CT2)
  [in10] -> M140/6(MR2)
  [in11] -> M140/7(T2)
  [in12] -> M140/8(EB2)
  [in13] -> M140/9(CT3)
  [in14] -> M140/10(F3)
  [in15] -> M140/11(E3)
  [in17] -> M140/12(T3)
  [in18] -> M140/13(EB3)
  M140/1(LL1) -> Eval139/1(In1)
  M140/2(LL2) -> Eval139/2(In2)
  M140/3(LL3) -> Eval139/3(In3)
  Eval139/1(Out1) -> To Workspace139/1
  [in1] -> M141/1(CT1)
  [in4] -> M141/2(MR1)
  [in5] -> M141/3(T1)
  [in6] -> M141/4(EB1)
  [in7] -> M141/5(CT2)
  [in10] -> M141/6(MR2)
  [in11] -> M141/7(T2)
  [in12] -> M141/8(EB2)
  [in13] -> M141/9(CT3)
  [in14] -> M141/10(F3)
  [in15] -> M141/11(E3)
  [in17] -> M141/12(T3)
  [in18] -> M141/13(EB3)
  M141/1(LL1) -> Eval140/1(In1)
  M141/2(LL2) -> Eval140/2(In2)
  M141/3(LL3) -> Eval140/3(In3)
  Eval140/1(Out1) -> To Workspace140/1
  [in1] -> M142/1(CT1)
  [in4] -> M142/2(MR1)
  [in5] -> M142/3(T1)
  [in6] -> M142/4(EB1)
  [in7] -> M142/5(CT2)
  [in10] -> M142/6(MR2)
  [in11] -> M142/7(T2)
  [in12] -> M142/8(EB2)
  [in13] -> M142/9(CT3)
  [in14] -> M142/10(F3)
  [in15] -> M142/11(E3)
  [in17] -> M142/12(T3)
  [in18] -> M142/13(EB3)
  M142/1(LL1) -> Eval141/1(In1)
  M142/2(LL2) -> Eval141/2(In2)
  M142/3(LL3) -> Eval141/3(In3)
  Eval141/1(Out1) -> To Workspace141/1
  [in1] -> M143/1(CT1)
  [in4] -> M143/2(MR1)
  [in5] -> M143/3(T1)
  [in6] -> M143/4(EB1)
  [in7] -> M143/5(CT2)
  [in10] -> M143/6(MR2)
  [in11] -> M143/7(T2)
  [in12] -> M143/8(EB2)
  [in13] -> M143/9(CT3)
  [in14] -> M143/10(F3)
  [in15] -> M143/11(E3)
  [in17] -> M143/12(T3)
  [in18] -> M143/13(EB3)
  M143/1(LL1) -> Eval142/1(In1)
  M143/2(LL2) -> Eval142/2(In2)
  M143/3(LL3) -> Eval142/3(In3)
  Eval142/1(Out1) -> To Workspace142/1
  [in1] -> M144/1(CT1)
  [in4] -> M144/2(MR1)
  [in5] -> M144/3(T1)
  [in6] -> M144/4(EB1)
  [in7] -> M144/5(CT2)
  [in10] -> M144/6(MR2)
  [in11] -> M144/7(T2)
  [in12] -> M144/8(EB2)
  [in13] -> M144/9(CT3)
  [in14] -> M144/10(F3)
  [in15] -> M144/11(E3)
  [in17] -> M144/12(T3)
  [in18] -> M144/13(EB3)
  M144/1(LL1) -> Eval143/1(In1)
  M144/2(LL2) -> Eval143/2(In2)
  M144/3(LL3) -> Eval143/3(In3)
  Eval143/1(Out1) -> To Workspace143/1
  [in1] -> M145/1(CT1)
  [in4] -> M145/2(MR1)
  [in5] -> M145/3(T1)
  [in6] -> M145/4(EB1)
  [in7] -> M145/5(CT2)
  [in10] -> M145/6(MR2)
  [in11] -> M145/7(T2)
  [in12] -> M145/8(EB2)
  [in13] -> M145/9(CT3)
  [in14] -> M145/10(F3)
  [in15] -> M145/11(E3)
  [in17] -> M145/12(T3)
  [in18] -> M145/13(EB3)
  M145/1(LL1) -> Eval144/1(In1)
  M145/2(LL2) -> Eval144/2(In2)
  M145/3(LL3) -> Eval144/3(In3)
  Eval144/1(Out1) -> To Workspace144/1
  [in1] -> M146/1(CT1)
  [in4] -> M146/2(MR1)
  [in5] -> M146/3(T1)
  [in6] -> M146/4(EB1)
  [in7] -> M146/5(CT2)
  [in10] -> M146/6(MR2)
  [in11] -> M146/7(T2)
  [in12] -> M146/8(EB2)
  [in13] -> M146/9(CT3)
  [in14] -> M146/10(F3)
  [in15] -> M146/11(E3)
  [in17] -> M146/12(T3)
  [in18] -> M146/13(EB3)
  M146/1(LL1) -> Eval145/1(In1)
  M146/2(LL2) -> Eval145/2(In2)
  M146/3(LL3) -> Eval145/3(In3)
  Eval145/1(Out1) -> To Workspace145/1
  [in1] -> M147/1(CT1)
  [in4] -> M147/2(MR1)
  [in5] -> M147/3(T1)
  [in6] -> M147/4(EB1)
  [in7] -> M147/5(CT2)
  [in10] -> M147/6(MR2)
  [in11] -> M147/7(T2)
  [in12] -> M147/8(EB2)
  [in13] -> M147/9(CT3)
  [in14] -> M147/10(F3)
  [in15] -> M147/11(E3)
  [in17] -> M147/12(T3)
  [in18] -> M147/13(EB3)
  M147/1(LL1) -> Eval146/1(In1)
  M147/2(LL2) -> Eval146/2(In2)
  M147/3(LL3) -> Eval146/3(In3)
  Eval146/1(Out1) -> To Workspace146/1
  [in1] -> M148/1(CT1)
  [in4] -> M148/2(MR1)
  [in5] -> M148/3(T1)
  [in6] -> M148/4(EB1)
  [in7] -> M148/5(CT2)
  [in10] -> M148/6(MR2)
  [in11] -> M148/7(T2)
  [in12] -> M148/8(EB2)
  [in13] -> M148/9(CT3)
  [in14] -> M148/10(F3)
  [in15] -> M148/11(E3)
  [in17] -> M148/12(T3)
  [in18] -> M148/13(EB3)
  M148/1(LL1) -> Eval147/1(In1)
  M148/2(LL2) -> Eval147/2(In2)
  M148/3(LL3) -> Eval147/3(In3)
  Eval147/1(Out1) -> To Workspace147/1
  [in1] -> M149/1(CT1)
  [in4] -> M149/2(MR1)
  [in5] -> M149/3(T1)
  [in6] -> M149/4(EB1)
  [in7] -> M149/5(CT2)
  [in10] -> M149/6(MR2)
  [in11] -> M149/7(T2)
  [in12] -> M149/8(EB2)
  [in13] -> M149/9(CT3)
  [in14] -> M149/10(F3)
  [in15] -> M149/11(E3)
  [in17] -> M149/12(T3)
  [in18] -> M149/13(EB3)
  M149/1(LL1) -> Eval148/1(In1)
  M149/2(LL2) -> Eval148/2(In2)
  M149/3(LL3) -> Eval148/3(In3)
  Eval148/1(Out1) -> To Workspace148/1
  [in1] -> M150/1(CT1)
  [in4] -> M150/2(MR1)
  [in5] -> M150/3(T1)
  [in6] -> M150/4(EB1)
  [in7] -> M150/5(CT2)
  [in10] -> M150/6(MR2)
  [in11] -> M150/7(T2)
  [in12] -> M150/8(EB2)
  [in13] -> M150/9(CT3)
  [in14] -> M150/10(F3)
  [in15] -> M150/11(E3)
  [in17] -> M150/12(T3)
  [in18] -> M150/13(EB3)
  M150/1(LL1) -> Eval149/1(In1)
  M150/2(LL2) -> Eval149/2(In2)
  M150/3(LL3) -> Eval149/3(In3)
  Eval149/1(Out1) -> To Workspace149/1
  [in1] -> M151/1(CT1)
  [in4] -> M151/2(MR1)
  [in5] -> M151/3(T1)
  [in6] -> M151/4(EB1)
  [in7] -> M151/5(CT2)
  [in10] -> M151/6(MR2)
  [in11] -> M151/7(T2)
  [in12] -> M151/8(EB2)
  [in13] -> M151/9(CT3)
  [in14] -> M151/10(F3)
  [in15] -> M151/11(E3)
  [in17] -> M151/12(T3)
  [in18] -> M151/13(EB3)
  M151/1(LL1) -> Eval150/1(In1)
  M151/2(LL2) -> Eval150/2(In2)
  M151/3(LL3) -> Eval150/3(In3)
  Eval150/1(Out1) -> To Workspace150/1
  [in1] -> M152/1(CT1)
  [in4] -> M152/2(MR1)
  [in5] -> M152/3(T1)
  [in6] -> M152/4(EB1)
  [in7] -> M152/5(CT2)
  [in10] -> M152/6(MR2)
  [in11] -> M152/7(T2)
  [in12] -> M152/8(EB2)
  [in13] -> M152/9(CT3)
  [in14] -> M152/10(F3)
  [in15] -> M152/11(E3)
  [in17] -> M152/12(T3)
  [in18] -> M152/13(EB3)
  M152/1(LL1) -> Eval151/1(In1)
  M152/2(LL2) -> Eval151/2(In2)
  M152/3(LL3) -> Eval151/3(In3)
  Eval151/1(Out1) -> To Workspace151/1
  [in1] -> M153/1(CT1)
  [in4] -> M153/2(MR1)
  [in5] -> M153/3(T1)
  [in6] -> M153/4(EB1)
  [in7] -> M153/5(CT2)
  [in10] -> M153/6(MR2)
  [in11] -> M153/7(T2)
  [in12] -> M153/8(EB2)
  [in13] -> M153/9(CT3)
  [in14] -> M153/10(F3)
  [in15] -> M153/11(E3)
  [in17] -> M153/12(T3)
  [in18] -> M153/13(EB3)
  M153/1(LL1) -> Eval152/1(In1)
  M153/2(LL2) -> Eval152/2(In2)
  M153/3(LL3) -> Eval152/3(In3)
  Eval152/1(Out1) -> To Workspace152/1
  [in1] -> M154/1(CT1)
  [in4] -> M154/2(MR1)
  [in5] -> M154/3(T1)
  [in6] -> M154/4(EB1)
  [in7] -> M154/5(CT2)
  [in10] -> M154/6(MR2)
  [in11] -> M154/7(T2)
  [in12] -> M154/8(EB2)
  [in13] -> M154/9(CT3)
  [in14] -> M154/10(F3)
  [in15] -> M154/11(E3)
  [in17] -> M154/12(T3)
  [in18] -> M154/13(EB3)
  M154/1(LL1) -> Eval153/1(In1)
  M154/2(LL2) -> Eval153/2(In2)
  M154/3(LL3) -> Eval153/3(In3)
  Eval153/1(Out1) -> To Workspace153/1
  [in1] -> M155/1(CT1)
  [in4] -> M155/2(MR1)
  [in5] -> M155/3(T1)
  [in6] -> M155/4(EB1)
  [in7] -> M155/5(CT2)
  [in10] -> M155/6(MR2)
  [in11] -> M155/7(T2)
  [in12] -> M155/8(EB2)
  [in13] -> M155/9(CT3)
  [in14] -> M155/10(F3)
  [in15] -> M155/11(E3)
  [in17] -> M155/12(T3)
  [in18] -> M155/13(EB3)
  M155/1(LL1) -> Eval154/1(In1)
  M155/2(LL2) -> Eval154/2(In2)
  M155/3(LL3) -> Eval154/3(In3)
  Eval154/1(Out1) -> To Workspace154/1
  [in1] -> M156/1(CT1)
  [in4] -> M156/2(MR1)
  [in5] -> M156/3(T1)
  [in6] -> M156/4(EB1)
  [in7] -> M156/5(CT2)
  [in10] -> M156/6(MR2)
  [in11] -> M156/7(T2)
  [in12] -> M156/8(EB2)
  [in13] -> M156/9(CT3)
  [in14] -> M156/10(F3)
  [in15] -> M156/11(E3)
  [in17] -> M156/12(T3)
  [in18] -> M156/13(EB3)
  M156/1(LL1) -> Eval155/1(In1)
  M156/2(LL2) -> Eval155/2(In2)
  M156/3(LL3) -> Eval155/3(In3)
  Eval155/1(Out1) -> To Workspace155/1
  [in1] -> M157/1(CT1)
  [in4] -> M157/2(MR1)
  [in5] -> M157/3(T1)
  [in6] -> M157/4(EB1)
  [in7] -> M157/5(CT2)
  [in10] -> M157/6(MR2)
  [in11] -> M157/7(T2)
  [in12] -> M157/8(EB2)
  [in13] -> M157/9(CT3)
  [in14] -> M157/10(F3)
  [in15] -> M157/11(E3)
  [in17] -> M157/12(T3)
  [in18] -> M157/13(EB3)
  M157/1(LL1) -> Eval156/1(In1)
  M157/2(LL2) -> Eval156/2(In2)
  M157/3(LL3) -> Eval156/3(In3)
  Eval156/1(Out1) -> To Workspace156/1
  [in1] -> M158/1(CT1)
  [in4] -> M158/2(MR1)
  [in5] -> M158/3(T1)
  [in6] -> M158/4(EB1)
  [in7] -> M158/5(CT2)
  [in10] -> M158/6(MR2)
  [in11] -> M158/7(T2)
  [in12] -> M158/8(EB2)
  [in13] -> M158/9(CT3)
  [in14] -> M158/10(F3)
  [in15] -> M158/11(E3)
  [in17] -> M158/12(T3)
  [in18] -> M158/13(EB3)
  M158/1(LL1) -> Eval157/1(In1)
  M158/2(LL2) -> Eval157/2(In2)
  M158/3(LL3) -> Eval157/3(In3)
  Eval157/1(Out1) -> To Workspace157/1
  [in1] -> M159/1(CT1)
  [in4] -> M159/2(MR1)
  [in5] -> M159/3(T1)
  [in6] -> M159/4(EB1)
  [in7] -> M159/5(CT2)
  [in10] -> M159/6(MR2)
  [in11] -> M159/7(T2)
  [in12] -> M159/8(EB2)
  [in13] -> M159/9(CT3)
  [in14] -> M159/10(F3)
  [in15] -> M159/11(E3)
  [in17] -> M159/12(T3)
  [in18] -> M159/13(EB3)
  M159/1(LL1) -> Eval158/1(In1)
  M159/2(LL2) -> Eval158/2(In2)
  M159/3(LL3) -> Eval158/3(In3)
  Eval158/1(Out1) -> To Workspace158/1
  [in1] -> M160/1(CT1)
  [in4] -> M160/2(MR1)
  [in5] -> M160/3(T1)
  [in6] -> M160/4(EB1)
  [in7] -> M160/5(CT2)
  [in10] -> M160/6(MR2)
  [in11] -> M160/7(T2)
  [in12] -> M160/8(EB2)
  [in13] -> M160/9(CT3)
  [in14] -> M160/10(F3)
  [in15] -> M160/11(E3)
  [in17] -> M160/12(T3)
  [in18] -> M160/13(EB3)
  M160/1(LL1) -> Eval159/1(In1)
  M160/2(LL2) -> Eval159/2(In2)
  M160/3(LL3) -> Eval159/3(In3)
  Eval159/1(Out1) -> To Workspace159/1
  [in1] -> M161/1(CT1)
  [in4] -> M161/2(MR1)
  [in5] -> M161/3(T1)
  [in6] -> M161/4(EB1)
  [in7] -> M161/5(CT2)
  [in10] -> M161/6(MR2)
  [in11] -> M161/7(T2)
  [in12] -> M161/8(EB2)
  [in13] -> M161/9(CT3)
  [in14] -> M161/10(F3)
  [in15] -> M161/11(E3)
  [in17] -> M161/12(T3)
  [in18] -> M161/13(EB3)
  M161/1(LL1) -> Eval160/1(In1)
  M161/2(LL2) -> Eval160/2(In2)
  M161/3(LL3) -> Eval160/3(In3)
  Eval160/1(Out1) -> To Workspace160/1
  [in1] -> M162/1(CT1)
  [in4] -> M162/2(MR1)
  [in5] -> M162/3(T1)
  [in6] -> M162/4(EB1)
  [in7] -> M162/5(CT2)
  [in10] -> M162/6(MR2)
  [in11] -> M162/7(T2)
  [in12] -> M162/8(EB2)
  [in13] -> M162/9(CT3)
  [in14] -> M162/10(F3)
  [in15] -> M162/11(E3)
  [in17] -> M162/12(T3)
  [in18] -> M162/13(EB3)
  M162/1(LL1) -> Eval161/1(In1)
  M162/2(LL2) -> Eval161/2(In2)
  M162/3(LL3) -> Eval161/3(In3)
  Eval161/1(Out1) -> To Workspace161/1
  [in1] -> M163/1(CT1)
  [in4] -> M163/2(MR1)
  [in5] -> M163/3(T1)
  [in6] -> M163/4(EB1)
  [in7] -> M163/5(CT2)
  [in10] -> M163/6(MR2)
  [in11] -> M163/7(T2)
  [in12] -> M163/8(EB2)
  [in13] -> M163/9(CT3)
  [in14] -> M163/10(F3)
  [in15] -> M163/11(E3)
  [in17] -> M163/12(T3)
  [in18] -> M163/13(EB3)
  M163/1(LL1) -> Eval162/1(In1)
  M163/2(LL2) -> Eval162/2(In2)
  M163/3(LL3) -> Eval162/3(In3)
  Eval162/1(Out1) -> To Workspace162/1
  [in1] -> M164/1(CT1)
  [in4] -> M164/2(MR1)
  [in5] -> M164/3(T1)
  [in6] -> M164/4(EB1)
  [in7] -> M164/5(CT2)
  [in10] -> M164/6(MR2)
  [in11] -> M164/7(T2)
  [in12] -> M164/8(EB2)
  [in13] -> M164/9(CT3)
  [in14] -> M164/10(F3)
  [in15] -> M164/11(E3)
  [in17] -> M164/12(T3)
  [in18] -> M164/13(EB3)
  M164/1(LL1) -> Eval163/1(In1)
  M164/2(LL2) -> Eval163/2(In2)
  M164/3(LL3) -> Eval163/3(In3)
  Eval163/1(Out1) -> To Workspace163/1
  [in1] -> M165/1(CT1)
  [in4] -> M165/2(MR1)
  [in5] -> M165/3(T1)
  [in6] -> M165/4(EB1)
  [in7] -> M165/5(CT2)
  [in10] -> M165/6(MR2)
  [in11] -> M165/7(T2)
  [in12] -> M165/8(EB2)
  [in13] -> M165/9(CT3)
  [in14] -> M165/10(F3)
  [in15] -> M165/11(E3)
  [in17] -> M165/12(T3)
  [in18] -> M165/13(EB3)
  M165/1(LL1) -> Eval164/1(In1)
  M165/2(LL2) -> Eval164/2(In2)
  M165/3(LL3) -> Eval164/3(In3)
  Eval164/1(Out1) -> To Workspace164/1
  [in1] -> M200/1(CT1)
  [in4] -> M200/2(MR1)
  [in5] -> M200/3(T1)
  [in6] -> M200/4(EB1)
  [in7] -> M200/5(CT2)
  [in10] -> M200/6(MR2)
  [in11] -> M200/7(T2)
  [in12] -> M200/8(EB2)
  [in13] -> M200/9(CT3)
  [in14] -> M200/10(F3)
  [in15] -> M200/11(E3)
  [in17] -> M200/12(T3)
  [in18] -> M200/13(EB3)
  M200/1(LL1) -> Eval199/1(In1)
  M200/2(LL2) -> Eval199/2(In2)
  M200/3(LL3) -> Eval199/3(In3)
  Eval199/1(Out1) -> To Workspace199/1
  [in1] -> M201/1(CT1)
  [in4] -> M201/2(MR1)
  [in5] -> M201/3(T1)
  [in6] -> M201/4(EB1)
  [in7] -> M201/5(CT2)
  [in10] -> M201/6(MR2)
  [in11] -> M201/7(T2)
  [in12] -> M201/8(EB2)
  [in13] -> M201/9(CT3)
  [in14] -> M201/10(F3)
  [in15] -> M201/11(E3)
  [in17] -> M201/12(T3)
  [in18] -> M201/13(EB3)
  M201/1(LL1) -> Eval200/1(In1)
  M201/2(LL2) -> Eval200/2(In2)
  M201/3(LL3) -> Eval200/3(In3)
  Eval200/1(Out1) -> To Workspace200/1
  [in1] -> M202/1(CT1)
  [in4] -> M202/2(MR1)
  [in5] -> M202/3(T1)
  [in6] -> M202/4(EB1)
  [in7] -> M202/5(CT2)
  [in10] -> M202/6(MR2)
  [in11] -> M202/7(T2)
  [in12] -> M202/8(EB2)
  [in13] -> M202/9(CT3)
  [in14] -> M202/10(F3)
  [in15] -> M202/11(E3)
  [in17] -> M202/12(T3)
  [in18] -> M202/13(EB3)
  M202/1(LL1) -> Eval201/1(In1)
  M202/2(LL2) -> Eval201/2(In2)
  M202/3(LL3) -> Eval201/3(In3)
  Eval201/1(Out1) -> To Workspace201/1
  [in1] -> M203/1(CT1)
  [in4] -> M203/2(MR1)
  [in5] -> M203/3(T1)
  [in6] -> M203/4(EB1)
  [in7] -> M203/5(CT2)
  [in10] -> M203/6(MR2)
  [in11] -> M203/7(T2)
  [in12] -> M203/8(EB2)
  [in13] -> M203/9(CT3)
  [in14] -> M203/10(F3)
  [in15] -> M203/11(E3)
  [in17] -> M203/12(T3)
  [in18] -> M203/13(EB3)
  M203/1(LL1) -> Eval202/1(In1)
  M203/2(LL2) -> Eval202/2(In2)
  M203/3(LL3) -> Eval202/3(In3)
  Eval202/1(Out1) -> To Workspace202/1
  [in1] -> M204/1(CT1)
  [in4] -> M204/2(MR1)
  [in5] -> M204/3(T1)
  [in6] -> M204/4(EB1)
  [in7] -> M204/5(CT2)
  [in10] -> M204/6(MR2)
  [in11] -> M204/7(T2)
  [in12] -> M204/8(EB2)
  [in13] -> M204/9(CT3)
  [in14] -> M204/10(F3)
  [in15] -> M204/11(E3)
  [in17] -> M204/12(T3)
  [in18] -> M204/13(EB3)
  M204/1(LL1) -> Eval203/1(In1)
  M204/2(LL2) -> Eval203/2(In2)
  M204/3(LL3) -> Eval203/3(In3)
  Eval203/1(Out1) -> To Workspace203/1
  [in1] -> M205/1(CT1)
  [in4] -> M205/2(MR1)
  [in5] -> M205/3(T1)
  [in6] -> M205/4(EB1)
  [in7] -> M205/5(CT2)
  [in10] -> M205/6(MR2)
  [in11] -> M205/7(T2)
  [in12] -> M205/8(EB2)
  [in13] -> M205/9(CT3)
  [in14] -> M205/10(F3)
  [in15] -> M205/11(E3)
  [in17] -> M205/12(T3)
  [in18] -> M205/13(EB3)
  M205/1(LL1) -> Eval204/1(In1)
  M205/2(LL2) -> Eval204/2(In2)
  M205/3(LL3) -> Eval204/3(In3)
  Eval204/1(Out1) -> To Workspace204/1
  [in1] -> M206/1(CT1)
  [in4] -> M206/2(MR1)
  [in5] -> M206/3(T1)
  [in6] -> M206/4(EB1)
  [in7] -> M206/5(CT2)
  [in10] -> M206/6(MR2)
  [in11] -> M206/7(T2)
  [in12] -> M206/8(EB2)
  [in13] -> M206/9(CT3)
  [in14] -> M206/10(F3)
  [in15] -> M206/11(E3)
  [in17] -> M206/12(T3)
  [in18] -> M206/13(EB3)
  M206/1(LL1) -> Eval205/1(In1)
  M206/2(LL2) -> Eval205/2(In2)
  M206/3(LL3) -> Eval205/3(In3)
  Eval205/1(Out1) -> To Workspace205/1
  [in1] -> M207/1(CT1)
  [in4] -> M207/2(MR1)
  [in5] -> M207/3(T1)
  [in6] -> M207/4(EB1)
  [in7] -> M207/5(CT2)
  [in10] -> M207/6(MR2)
  [in11] -> M207/7(T2)
  [in12] -> M207/8(EB2)
  [in13] -> M207/9(CT3)
  [in14] -> M207/10(F3)
  [in15] -> M207/11(E3)
  [in17] -> M207/12(T3)
  [in18] -> M207/13(EB3)
  M207/1(LL1) -> Eval206/1(In1)
  M207/2(LL2) -> Eval206/2(In2)
  M207/3(LL3) -> Eval206/3(In3)
  Eval206/1(Out1) -> To Workspace206/1
  [in1] -> M208/1(CT1)
  [in4] -> M208/2(MR1)
  [in5] -> M208/3(T1)
  [in6] -> M208/4(EB1)
  [in7] -> M208/5(CT2)
  [in10] -> M208/6(MR2)
  [in11] -> M208/7(T2)
  [in12] -> M208/8(EB2)
  [in13] -> M208/9(CT3)
  [in14] -> M208/10(F3)
  [in15] -> M208/11(E3)
  [in17] -> M208/12(T3)
  [in18] -> M208/13(EB3)
  M208/1(LL1) -> Eval207/1(In1)
  M208/2(LL2) -> Eval207/2(In2)
  M208/3(LL3) -> Eval207/3(In3)
  Eval207/1(Out1) -> To Workspace207/1
  [in1] -> M209/1(CT1)
  [in4] -> M209/2(MR1)
  [in5] -> M209/3(T1)
  [in6] -> M209/4(EB1)
  [in7] -> M209/5(CT2)
  [in10] -> M209/6(MR2)
  [in11] -> M209/7(T2)
  [in12] -> M209/8(EB2)
  [in13] -> M209/9(CT3)
  [in14] -> M209/10(F3)
  [in15] -> M209/11(E3)
  [in17] -> M209/12(T3)
  [in18] -> M209/13(EB3)
  M209/1(LL1) -> Eval208/1(In1)
  M209/2(LL2) -> Eval208/2(In2)
  M209/3(LL3) -> Eval208/3(In3)
  Eval208/1(Out1) -> To Workspace208/1
  [in1] -> M222/1(CT1)
  [in4] -> M222/2(MR1)
  [in5] -> M222/3(T1)
  [in6] -> M222/4(EB1)
  [in7] -> M222/5(CT2)
  [in10] -> M222/6(MR2)
  [in11] -> M222/7(T2)
  [in12] -> M222/8(EB2)
  [in13] -> M222/9(CT3)
  [in14] -> M222/10(F3)
  [in15] -> M222/11(E3)
  [in17] -> M222/12(T3)
  [in18] -> M222/13(EB3)
  M222/1(LL1) -> Eval221/1(In1)
  M222/2(LL2) -> Eval221/2(In2)
  M222/3(LL3) -> Eval221/3(In3)
  Eval221/1(Out1) -> To Workspace221/1
  [in1] -> M223/1(CT1)
  [in4] -> M223/2(MR1)
  [in5] -> M223/3(T1)
  [in6] -> M223/4(EB1)
  [in7] -> M223/5(CT2)
  [in10] -> M223/6(MR2)
  [in11] -> M223/7(T2)
  [in12] -> M223/8(EB2)
  [in13] -> M223/9(CT3)
  [in14] -> M223/10(F3)
  [in15] -> M223/11(E3)
  [in17] -> M223/12(T3)
  [in18] -> M223/13(EB3)
  M223/1(LL1) -> Eval222/1(In1)
  M223/2(LL2) -> Eval222/2(In2)
  M223/3(LL3) -> Eval222/3(In3)
  Eval222/1(Out1) -> To Workspace222/1
  [in1] -> M224/1(CT1)
  [in4] -> M224/2(MR1)
  [in5] -> M224/3(T1)
  [in6] -> M224/4(EB1)
  [in7] -> M224/5(CT2)
  [in10] -> M224/6(MR2)
  [in11] -> M224/7(T2)
  [in12] -> M224/8(EB2)
  [in13] -> M224/9(CT3)
  [in14] -> M224/10(F3)
  [in15] -> M224/11(E3)
  [in17] -> M224/12(T3)
  [in18] -> M224/13(EB3)
  M224/1(LL1) -> Eval223/1(In1)
  M224/2(LL2) -> Eval223/2(In2)
  M224/3(LL3) -> Eval223/3(In3)
  Eval223/1(Out1) -> To Workspace223/1
  [in1] -> M225/1(CT1)
  [in4] -> M225/2(MR1)
  [in5] -> M225/3(T1)
  [in6] -> M225/4(EB1)
  [in7] -> M225/5(CT2)
  [in10] -> M225/6(MR2)
  [in11] -> M225/7(T2)
  [in12] -> M225/8(EB2)
  [in13] -> M225/9(CT3)
  [in14] -> M225/10(F3)
  [in15] -> M225/11(E3)
  [in17] -> M225/12(T3)
  [in18] -> M225/13(EB3)
  M225/1(LL1) -> Eval224/1(In1)
  M225/2(LL2) -> Eval224/2(In2)
  M225/3(LL3) -> Eval224/3(In3)
  Eval224/1(Out1) -> To Workspace224/1
  [in1] -> M226/1(CT1)
  [in4] -> M226/2(MR1)
  [in5] -> M226/3(T1)
  [in6] -> M226/4(EB1)
  [in7] -> M226/5(CT2)
  [in10] -> M226/6(MR2)
  [in11] -> M226/7(T2)
  [in12] -> M226/8(EB2)
  [in13] -> M226/9(CT3)
  [in14] -> M226/10(F3)
  [in15] -> M226/11(E3)
  [in17] -> M226/12(T3)
  [in18] -> M226/13(EB3)
  M226/1(LL1) -> Eval225/1(In1)
  M226/2(LL2) -> Eval225/2(In2)
  M226/3(LL3) -> Eval225/3(In3)
  Eval225/1(Out1) -> To Workspace225/1
  [in1] -> M227/1(CT1)
  [in4] -> M227/2(MR1)
  [in5] -> M227/3(T1)
  [in6] -> M227/4(EB1)
  [in7] -> M227/5(CT2)
  [in10] -> M227/6(MR2)
  [in11] -> M227/7(T2)
  [in12] -> M227/8(EB2)
  [in13] -> M227/9(CT3)
  [in14] -> M227/10(F3)
  [in15] -> M227/11(E3)
  [in17] -> M227/12(T3)
  [in18] -> M227/13(EB3)
  M227/1(LL1) -> Eval226/1(In1)
  M227/2(LL2) -> Eval226/2(In2)
  M227/3(LL3) -> Eval226/3(In3)
  Eval226/1(Out1) -> To Workspace226/1
  [in1] -> M228/1(CT1)
  [in4] -> M228/2(MR1)
  [in5] -> M228/3(T1)
  [in6] -> M228/4(EB1)
  [in7] -> M228/5(CT2)
  [in10] -> M228/6(MR2)
  [in11] -> M228/7(T2)
  [in12] -> M228/8(EB2)
  [in13] -> M228/9(CT3)
  [in14] -> M228/10(F3)
  [in15] -> M228/11(E3)
  [in17] -> M228/12(T3)
  [in18] -> M228/13(EB3)
  M228/1(LL1) -> Eval227/1(In1)
  M228/2(LL2) -> Eval227/2(In2)
  M228/3(LL3) -> Eval227/3(In3)
  Eval227/1(Out1) -> To Workspace227/1
  [in1] -> M229/1(CT1)
  [in4] -> M229/2(MR1)
  [in5] -> M229/3(T1)
  [in6] -> M229/4(EB1)
  [in7] -> M229/5(CT2)
  [in10] -> M229/6(MR2)
  [in11] -> M229/7(T2)
  [in12] -> M229/8(EB2)
  [in13] -> M229/9(CT3)
  [in14] -> M229/10(F3)
  [in15] -> M229/11(E3)
  [in17] -> M229/12(T3)
  [in18] -> M229/13(EB3)
  M229/1(LL1) -> Eval228/1(In1)
  M229/2(LL2) -> Eval228/2(In2)
  M229/3(LL3) -> Eval228/3(In3)
  Eval228/1(Out1) -> To Workspace228/1
  [in1] -> M230/1(CT1)
  [in4] -> M230/2(MR1)
  [in5] -> M230/3(T1)
  [in6] -> M230/4(EB1)
  [in7] -> M230/5(CT2)
  [in10] -> M230/6(MR2)
  [in11] -> M230/7(T2)
  [in12] -> M230/8(EB2)
  [in13] -> M230/9(CT3)
  [in14] -> M230/10(F3)
  [in15] -> M230/11(E3)
  [in17] -> M230/12(T3)
  [in18] -> M230/13(EB3)
  M230/1(LL1) -> Eval229/1(In1)
  M230/2(LL2) -> Eval229/2(In2)
  M230/3(LL3) -> Eval229/3(In3)
  Eval229/1(Out1) -> To Workspace229/1
  [in1] -> M231/1(CT1)
  [in4] -> M231/2(MR1)
  [in5] -> M231/3(T1)
  [in6] -> M231/4(EB1)
  [in7] -> M231/5(CT2)
  [in10] -> M231/6(MR2)
  [in11] -> M231/7(T2)
  [in12] -> M231/8(EB2)
  [in13] -> M231/9(CT3)
  [in14] -> M231/10(F3)
  [in15] -> M231/11(E3)
  [in17] -> M231/12(T3)
  [in18] -> M231/13(EB3)
  M231/1(LL1) -> Eval230/1(In1)
  M231/2(LL2) -> Eval230/2(In2)
  M231/3(LL3) -> Eval230/3(In3)
  Eval230/1(Out1) -> To Workspace230/1
  [in1] -> M232/1(CT1)
  [in4] -> M232/2(MR1)
  [in5] -> M232/3(T1)
  [in6] -> M232/4(EB1)
  [in7] -> M232/5(CT2)
  [in10] -> M232/6(MR2)
  [in11] -> M232/7(T2)
  [in12] -> M232/8(EB2)
  [in13] -> M232/9(CT3)
  [in14] -> M232/10(F3)
  [in15] -> M232/11(E3)
  [in17] -> M232/12(T3)
  [in18] -> M232/13(EB3)
  M232/1(LL1) -> Eval231/1(In1)
  M232/2(LL2) -> Eval231/2(In2)
  M232/3(LL3) -> Eval231/3(In3)
  Eval231/1(Out1) -> To Workspace231/1
  [in1] -> M233/1(CT1)
  [in4] -> M233/2(MR1)
  [in5] -> M233/3(T1)
  [in6] -> M233/4(EB1)
  [in7] -> M233/5(CT2)
  [in10] -> M233/6(MR2)
  [in11] -> M233/7(T2)
  [in12] -> M233/8(EB2)
  [in13] -> M233/9(CT3)
  [in14] -> M233/10(F3)
  [in15] -> M233/11(E3)
  [in17] -> M233/12(T3)
  [in18] -> M233/13(EB3)
  M233/1(LL1) -> Eval232/1(In1)
  M233/2(LL2) -> Eval232/2(In2)
  M233/3(LL3) -> Eval232/3(In3)
  Eval232/1(Out1) -> To Workspace232/1
  [in1] -> M234/1(CT1)
  [in4] -> M234/2(MR1)
  [in5] -> M234/3(T1)
  [in6] -> M234/4(EB1)
  [in7] -> M234/5(CT2)
  [in10] -> M234/6(MR2)
  [in11] -> M234/7(T2)
  [in12] -> M234/8(EB2)
  [in13] -> M234/9(CT3)
  [in14] -> M234/10(F3)
  [in15] -> M234/11(E3)
  [in17] -> M234/12(T3)
  [in18] -> M234/13(EB3)
  M234/1(LL1) -> Eval233/1(In1)
  M234/2(LL2) -> Eval233/2(In2)
  M234/3(LL3) -> Eval233/3(In3)
  Eval233/1(Out1) -> To Workspace233/1
  [in1] -> M235/1(CT1)
  [in4] -> M235/2(MR1)
  [in5] -> M235/3(T1)
  [in6] -> M235/4(EB1)
  [in7] -> M235/5(CT2)
  [in10] -> M235/6(MR2)
  [in11] -> M235/7(T2)
  [in12] -> M235/8(EB2)
  [in13] -> M235/9(CT3)
  [in14] -> M235/10(F3)
  [in15] -> M235/11(E3)
  [in17] -> M235/12(T3)
  [in18] -> M235/13(EB3)
  M235/1(LL1) -> Eval234/1(In1)
  M235/2(LL2) -> Eval234/2(In2)
  M235/3(LL3) -> Eval234/3(In3)
  Eval234/1(Out1) -> To Workspace234/1
  [in1] -> M236/1(CT1)
  [in4] -> M236/2(MR1)
  [in5] -> M236/3(T1)
  [in6] -> M236/4(EB1)
  [in7] -> M236/5(CT2)
  [in10] -> M236/6(MR2)
  [in11] -> M236/7(T2)
  [in12] -> M236/8(EB2)
  [in13] -> M236/9(CT3)
  [in14] -> M236/10(F3)
  [in15] -> M236/11(E3)
  [in17] -> M236/12(T3)
  [in18] -> M236/13(EB3)
  M236/1(LL1) -> Eval235/1(In1)
  M236/2(LL2) -> Eval235/2(In2)
  M236/3(LL3) -> Eval235/3(In3)
  Eval235/1(Out1) -> To Workspace235/1
  [in1] -> M237/1(CT1)
  [in4] -> M237/2(MR1)
  [in5] -> M237/3(T1)
  [in6] -> M237/4(EB1)
  [in7] -> M237/5(CT2)
  [in10] -> M237/6(MR2)
  [in11] -> M237/7(T2)
  [in12] -> M237/8(EB2)
  [in13] -> M237/9(CT3)
  [in14] -> M237/10(F3)
  [in15] -> M237/11(E3)
  [in17] -> M237/12(T3)
  [in18] -> M237/13(EB3)
  M237/1(LL1) -> Eval236/1(In1)
  M237/2(LL2) -> Eval236/2(In2)
  M237/3(LL3) -> Eval236/3(In3)
  Eval236/1(Out1) -> To Workspace236/1
  [in1] -> M238/1(CT1)
  [in4] -> M238/2(MR1)
  [in5] -> M238/3(T1)
  [in6] -> M238/4(EB1)
  [in7] -> M238/5(CT2)
  [in10] -> M238/6(MR2)
  [in11] -> M238/7(T2)
  [in12] -> M238/8(EB2)
  [in13] -> M238/9(CT3)
  [in14] -> M238/10(F3)
  [in15] -> M238/11(E3)
  [in17] -> M238/12(T3)
  [in18] -> M238/13(EB3)
  M238/1(LL1) -> Eval237/1(In1)
  M238/2(LL2) -> Eval237/2(In2)
  M238/3(LL3) -> Eval237/3(In3)
  Eval237/1(Out1) -> To Workspace237/1
  [in1] -> M239/1(CT1)
  [in4] -> M239/2(MR1)
  [in5] -> M239/3(T1)
  [in6] -> M239/4(EB1)
  [in7] -> M239/5(CT2)
  [in10] -> M239/6(MR2)
  [in11] -> M239/7(T2)
  [in12] -> M239/8(EB2)
  [in13] -> M239/9(CT3)
  [in14] -> M239/10(F3)
  [in15] -> M239/11(E3)
  [in17] -> M239/12(T3)
  [in18] -> M239/13(EB3)
  M239/1(LL1) -> Eval238/1(In1)
  M239/2(LL2) -> Eval238/2(In2)
  M239/3(LL3) -> Eval238/3(In3)
  Eval238/1(Out1) -> To Workspace238/1
  [in1] -> M240/1(CT1)
  [in4] -> M240/2(MR1)
  [in5] -> M240/3(T1)
  [in6] -> M240/4(EB1)
  [in7] -> M240/5(CT2)
  [in10] -> M240/6(MR2)
  [in11] -> M240/7(T2)
  [in12] -> M240/8(EB2)
  [in13] -> M240/9(CT3)
  [in14] -> M240/10(F3)
  [in15] -> M240/11(E3)
  [in17] -> M240/12(T3)
  [in18] -> M240/13(EB3)
  M240/1(LL1) -> Eval239/1(In1)
  M240/2(LL2) -> Eval239/2(In2)
  M240/3(LL3) -> Eval239/3(In3)
  Eval239/1(Out1) -> To Workspace239/1
  [in1] -> M241/1(CT1)
  [in4] -> M241/2(MR1)
  [in5] -> M241/3(T1)
  [in6] -> M241/4(EB1)
  [in7] -> M241/5(CT2)
  [in10] -> M241/6(MR2)
  [in11] -> M241/7(T2)
  [in12] -> M241/8(EB2)
  [in13] -> M241/9(CT3)
  [in14] -> M241/10(F3)
  [in15] -> M241/11(E3)
  [in17] -> M241/12(T3)
  [in18] -> M241/13(EB3)
  M241/1(LL1) -> Eval240/1(In1)
  M241/2(LL2) -> Eval240/2(In2)
  M241/3(LL3) -> Eval240/3(In3)
  Eval240/1(Out1) -> To Workspace240/1
  [in1] -> M242/1(CT1)
  [in4] -> M242/2(MR1)
  [in5] -> M242/3(T1)
  [in6] -> M242/4(EB1)
  [in7] -> M242/5(CT2)
  [in10] -> M242/6(MR2)
  [in11] -> M242/7(T2)
  [in12] -> M242/8(EB2)
  [in13] -> M242/9(CT3)
  [in14] -> M242/10(F3)
  [in15] -> M242/11(E3)
  [in17] -> M242/12(T3)
  [in18] -> M242/13(EB3)
  M242/1(LL1) -> Eval241/1(In1)
  M242/2(LL2) -> Eval241/2(In2)
  M242/3(LL3) -> Eval241/3(In3)
  Eval241/1(Out1) -> To Workspace241/1
  [in1] -> M243/1(CT1)
  [in4] -> M243/2(MR1)
  [in5] -> M243/3(T1)
  [in6] -> M243/4(EB1)
  [in7] -> M243/5(CT2)
  [in10] -> M243/6(MR2)
  [in11] -> M243/7(T2)
  [in12] -> M243/8(EB2)
  [in13] -> M243/9(CT3)
  [in14] -> M243/10(F3)
  [in15] -> M243/11(E3)
  [in17] -> M243/12(T3)
  [in18] -> M243/13(EB3)
  M243/1(LL1) -> Eval242/1(In1)
  M243/2(LL2) -> Eval242/2(In2)
  M243/3(LL3) -> Eval242/3(In3)
  Eval242/1(Out1) -> To Workspace242/1
  [in1] -> M244/1(CT1)
  [in4] -> M244/2(MR1)
  [in5] -> M244/3(T1)
  [in6] -> M244/4(EB1)
  [in7] -> M244/5(CT2)
  [in10] -> M244/6(MR2)
  [in11] -> M244/7(T2)
  [in12] -> M244/8(EB2)
  [in13] -> M244/9(CT3)
  [in14] -> M244/10(F3)
  [in15] -> M244/11(E3)
  [in17] -> M244/12(T3)
  [in18] -> M244/13(EB3)
  M244/1(LL1) -> Eval243/1(In1)
  M244/2(LL2) -> Eval243/2(In2)
  M244/3(LL3) -> Eval243/3(In3)
  Eval243/1(Out1) -> To Workspace243/1
  [in1] -> M245/1(CT1)
  [in4] -> M245/2(MR1)
  [in5] -> M245/3(T1)
  [in6] -> M245/4(EB1)
  [in7] -> M245/5(CT2)
  [in10] -> M245/6(MR2)
  [in11] -> M245/7(T2)
  [in12] -> M245/8(EB2)
  [in13] -> M245/9(CT3)
  [in14] -> M245/10(F3)
  [in15] -> M245/11(E3)
  [in17] -> M245/12(T3)
  [in18] -> M245/13(EB3)
  M245/1(LL1) -> Eval244/1(In1)
  M245/2(LL2) -> Eval244/2(In2)
  M245/3(LL3) -> Eval244/3(In3)
  Eval244/1(Out1) -> To Workspace244/1
  [in1] -> M246/1(CT1)
  [in4] -> M246/2(MR1)
  [in5] -> M246/3(T1)
  [in6] -> M246/4(EB1)
  [in7] -> M246/5(CT2)
  [in10] -> M246/6(MR2)
  [in11] -> M246/7(T2)
  [in12] -> M246/8(EB2)
  [in13] -> M246/9(CT3)
  [in14] -> M246/10(F3)
  [in15] -> M246/11(E3)
  [in17] -> M246/12(T3)
  [in18] -> M246/13(EB3)
  M246/1(LL1) -> Eval245/1(In1)
  M246/2(LL2) -> Eval245/2(In2)
  M246/3(LL3) -> Eval245/3(In3)
  Eval245/1(Out1) -> To Workspace245/1
  Inputs/1(CT1) -> dtc_CT1/1
  dtc_CT1/1 -> CPSUT/1(CT1), [in1]
  Inputs/2(MR1) -> dtc_MR1/1
  dtc_MR1/1 -> CPSUT/2(MR1), [in4]
  Inputs/3(T1) -> dtc_T1/1
  dtc_T1/1 -> CPSUT/3(T1), [in5]
  Inputs/4(EB1) -> dtc_EB1/1
  dtc_EB1/1 -> CPSUT/4(EB1), [in6]
  Inputs/5(CT2) -> dtc_CT2/1
  dtc_CT2/1 -> CPSUT/5(CT2), [in7]
  Inputs/6(MR2) -> dtc_MR2/1
  dtc_MR2/1 -> CPSUT/6(MR2), [in10]
  Inputs/7(T2) -> dtc_T2/1
  dtc_T2/1 -> CPSUT/7(T2), [in11]
  Inputs/8(EB2) -> dtc_EB2/1
  dtc_EB2/1 -> CPSUT/8(EB2), [in12]
  Inputs/9(CT3) -> dtc_CT3/1
  dtc_CT3/1 -> CPSUT/9(CT3), [in13]
  Inputs/10(F3) -> dtc_F3/1
  dtc_F3/1 -> CPSUT/10(F3), [in14]
  Inputs/11(E3) -> dtc_E3/1
  dtc_E3/1 -> CPSUT/11(E3), [in15]
  Inputs/12(T3) -> dtc_T3/1
  dtc_T3/1 -> CPSUT/12(T3), [in17]
  Inputs/13(EB3) -> dtc_EB3/1
  dtc_EB3/1 -> CPSUT/13(EB3), [in18]
